simulink model "model"  (R2014a)
(part 4 of 6)

  bus259 : powerlib/Measurements/Load Flow Bus  LConnTagsString=a  ID=bus259  Vbase=440000  Vref=1  Vangle=0  VLF=1  angleLF=0
      settings: AttributesFormatString=|
      | %<ID>
      | %<Vbase>V
      | %<VLF>pu
      | %<angleLF>deg.
      | %<Name>
  bus26 : powerlib/Measurements/Load Flow Bus  LConnTagsString=a  ID=bus26  Vbase=138000  Vref=1  Vangle=0  VLF=1  angleLF=0
      settings: AttributesFormatString=|
      | %<ID>
      | %<Vbase>V
      | %<VLF>pu
      | %<angleLF>deg.
      | %<Name>
  bus260 : powerlib/Measurements/Load Flow Bus  LConnTagsString=a  ID=bus260  Vbase=440000  Vref=1  Vangle=0  VLF=1  angleLF=0
      settings: AttributesFormatString=|
      | %<ID>
      | %<Vbase>V
      | %<VLF>pu
      | %<angleLF>deg.
      | %<Name>
  bus261 : powerlib/Measurements/Load Flow Bus  LConnTagsString=a  ID=bus261  Vbase=440000  Vref=1  Vangle=0  VLF=1  angleLF=0
      settings: AttributesFormatString=|
      | %<ID>
      | %<Vbase>V
      | %<VLF>pu
      | %<angleLF>deg.
      | %<Name>
  bus262 : powerlib/Measurements/Load Flow Bus  LConnTagsString=a  ID=bus262  Vbase=500000  Vref=1  Vangle=0  VLF=1  angleLF=0
      settings: AttributesFormatString=|
      | %<ID>
      | %<Vbase>V
      | %<VLF>pu
      | %<angleLF>deg.
      | %<Name>
  bus263 : powerlib/Measurements/Load Flow Bus  LConnTagsString=a  ID=bus263  Vbase=500000  Vref=1  Vangle=0  VLF=1  angleLF=0
      settings: AttributesFormatString=|
      | %<ID>
      | %<Vbase>V
      | %<VLF>pu
      | %<angleLF>deg.
      | %<Name>
  bus264 : powerlib/Measurements/Load Flow Bus  LConnTagsString=a  ID=bus264  Vbase=500000  Vref=1  Vangle=0  VLF=1  angleLF=0
      settings: AttributesFormatString=|
      | %<ID>
      | %<Vbase>V
      | %<VLF>pu
      | %<angleLF>deg.
      | %<Name>
  bus265 : powerlib/Measurements/Load Flow Bus  LConnTagsString=a  ID=bus265  Vbase=500000  Vref=1  Vangle=0  VLF=1  angleLF=0
      settings: AttributesFormatString=|
      | %<ID>
      | %<Vbase>V
      | %<VLF>pu
      | %<angleLF>deg.
      | %<Name>
  bus266 : powerlib/Measurements/Load Flow Bus  LConnTagsString=a  ID=bus266  Vbase=500000  Vref=1  Vangle=0  VLF=1  angleLF=0
      settings: AttributesFormatString=|
      | %<ID>
      | %<Vbase>V
      | %<VLF>pu
      | %<angleLF>deg.
      | %<Name>
  bus267 : powerlib/Measurements/Load Flow Bus  LConnTagsString=a  ID=bus267  Vbase=500000  Vref=1  Vangle=0  VLF=1  angleLF=0
      settings: AttributesFormatString=|
      | %<ID>
      | %<Vbase>V
      | %<VLF>pu
      | %<angleLF>deg.
      | %<Name>
  bus268 : powerlib/Measurements/Load Flow Bus  LConnTagsString=a  ID=bus268  Vbase=500000  Vref=1  Vangle=0  VLF=1  angleLF=0
      settings: AttributesFormatString=|
      | %<ID>
      | %<Vbase>V
      | %<VLF>pu
      | %<angleLF>deg.
      | %<Name>
  bus269 : powerlib/Measurements/Load Flow Bus  LConnTagsString=a  ID=bus269  Vbase=500000  Vref=1  Vangle=0  VLF=1  angleLF=0
      settings: AttributesFormatString=|
      | %<ID>
      | %<Vbase>V
      | %<VLF>pu
      | %<angleLF>deg.
      | %<Name>
  bus27 : powerlib/Measurements/Load Flow Bus  LConnTagsString=a  ID=bus27  Vbase=138000  Vref=1  Vangle=0  VLF=1  angleLF=0
      settings: AttributesFormatString=|
      | %<ID>
      | %<Vbase>V
      | %<VLF>pu
      | %<angleLF>deg.
      | %<Name>
  bus270 : powerlib/Measurements/Load Flow Bus  LConnTagsString=a  ID=bus270  Vbase=500000  Vref=1  Vangle=0  VLF=1  angleLF=0
      settings: AttributesFormatString=|
      | %<ID>
      | %<Vbase>V
      | %<VLF>pu
      | %<angleLF>deg.
      | %<Name>
  bus271 : powerlib/Measurements/Load Flow Bus  LConnTagsString=a  ID=bus271  Vbase=500000  Vref=1  Vangle=0  VLF=1  angleLF=0
      settings: AttributesFormatString=|
      | %<ID>
      | %<Vbase>V
      | %<VLF>pu
      | %<angleLF>deg.
      | %<Name>
  bus272 : powerlib/Measurements/Load Flow Bus  LConnTagsString=a  ID=bus272  Vbase=500000  Vref=1  Vangle=0  VLF=1  angleLF=0
      settings: AttributesFormatString=|
      | %<ID>
      | %<Vbase>V
      | %<VLF>pu
      | %<angleLF>deg.
      | %<Name>
  bus273 : powerlib/Measurements/Load Flow Bus  LConnTagsString=a  ID=bus273  Vbase=500000  Vref=1  Vangle=0  VLF=1  angleLF=0
      settings: AttributesFormatString=|
      | %<ID>
      | %<Vbase>V
      | %<VLF>pu
      | %<angleLF>deg.
      | %<Name>
  bus274 : powerlib/Measurements/Load Flow Bus  LConnTagsString=a  ID=bus274  Vbase=500000  Vref=1  Vangle=0  VLF=1  angleLF=0
      settings: AttributesFormatString=|
      | %<ID>
      | %<Vbase>V
      | %<VLF>pu
      | %<angleLF>deg.
      | %<Name>
  bus275 : powerlib/Measurements/Load Flow Bus  LConnTagsString=a  ID=bus275  Vbase=500000  Vref=1  Vangle=0  VLF=1  angleLF=0
      settings: AttributesFormatString=|
      | %<ID>
      | %<Vbase>V
      | %<VLF>pu
      | %<angleLF>deg.
      | %<Name>
  bus276 : powerlib/Measurements/Load Flow Bus  LConnTagsString=a  ID=bus276  Vbase=500000  Vref=1  Vangle=0  VLF=1  angleLF=0
      settings: AttributesFormatString=|
      | %<ID>
      | %<Vbase>V
      | %<VLF>pu
      | %<angleLF>deg.
      | %<Name>
  bus277 : powerlib/Measurements/Load Flow Bus  LConnTagsString=a  ID=bus277  Vbase=500000  Vref=1  Vangle=0  VLF=1  angleLF=0
      settings: AttributesFormatString=|
      | %<ID>
      | %<Vbase>V
      | %<VLF>pu
      | %<angleLF>deg.
      | %<Name>
  bus278 : powerlib/Measurements/Load Flow Bus  LConnTagsString=a  ID=bus278  Vbase=500000  Vref=1  Vangle=0  VLF=1  angleLF=0
      settings: AttributesFormatString=|
      | %<ID>
      | %<Vbase>V
      | %<VLF>pu
      | %<angleLF>deg.
      | %<Name>
  bus279 : powerlib/Measurements/Load Flow Bus  LConnTagsString=a  ID=bus279  Vbase=500000  Vref=1  Vangle=0  VLF=1  angleLF=0
      settings: AttributesFormatString=|
      | %<ID>
      | %<Vbase>V
      | %<VLF>pu
      | %<angleLF>deg.
      | %<Name>
  bus28 : powerlib/Measurements/Load Flow Bus  LConnTagsString=a  ID=bus28  Vbase=138000  Vref=1  Vangle=0  VLF=1  angleLF=0
      settings: AttributesFormatString=|
      | %<ID>
      | %<Vbase>V
      | %<VLF>pu
      | %<angleLF>deg.
      | %<Name>
  bus280 : powerlib/Measurements/Load Flow Bus  LConnTagsString=a  ID=bus280  Vbase=500000  Vref=1  Vangle=0  VLF=1  angleLF=0
      settings: AttributesFormatString=|
      | %<ID>
      | %<Vbase>V
      | %<VLF>pu
      | %<angleLF>deg.
      | %<Name>
  bus281 : powerlib/Measurements/Load Flow Bus  LConnTagsString=a  ID=bus281  Vbase=500000  Vref=1  Vangle=0  VLF=1  angleLF=0
      settings: AttributesFormatString=|
      | %<ID>
      | %<Vbase>V
      | %<VLF>pu
      | %<angleLF>deg.
      | %<Name>
  bus282 : powerlib/Measurements/Load Flow Bus  LConnTagsString=a  ID=bus282  Vbase=500000  Vref=1  Vangle=0  VLF=1  angleLF=0
      settings: AttributesFormatString=|
      | %<ID>
      | %<Vbase>V
      | %<VLF>pu
      | %<angleLF>deg.
      | %<Name>
  bus283 : powerlib/Measurements/Load Flow Bus  LConnTagsString=a  ID=bus283  Vbase=500000  Vref=1  Vangle=0  VLF=1  angleLF=0
      settings: AttributesFormatString=|
      | %<ID>
      | %<Vbase>V
      | %<VLF>pu
      | %<angleLF>deg.
      | %<Name>
  bus284 : powerlib/Measurements/Load Flow Bus  LConnTagsString=a  ID=bus284  Vbase=500000  Vref=1  Vangle=0  VLF=1  angleLF=0
      settings: AttributesFormatString=|
      | %<ID>
      | %<Vbase>V
      | %<VLF>pu
      | %<angleLF>deg.
      | %<Name>
  bus285 : powerlib/Measurements/Load Flow Bus  LConnTagsString=a  ID=bus285  Vbase=500000  Vref=1  Vangle=0  VLF=1  angleLF=0
      settings: AttributesFormatString=|
      | %<ID>
      | %<Vbase>V
      | %<VLF>pu
      | %<angleLF>deg.
      | %<Name>
  bus286 : powerlib/Measurements/Load Flow Bus  LConnTagsString=a  ID=bus286  Vbase=500000  Vref=1  Vangle=0  VLF=1  angleLF=0
      settings: AttributesFormatString=|
      | %<ID>
      | %<Vbase>V
      | %<VLF>pu
      | %<angleLF>deg.
      | %<Name>
  bus287 : powerlib/Measurements/Load Flow Bus  LConnTagsString=a  ID=bus287  Vbase=500000  Vref=1  Vangle=0  VLF=1  angleLF=0
      settings: AttributesFormatString=|
      | %<ID>
      | %<Vbase>V
      | %<VLF>pu
      | %<angleLF>deg.
      | %<Name>
  bus288 : powerlib/Measurements/Load Flow Bus  LConnTagsString=a  ID=bus288  Vbase=500000  Vref=1  Vangle=0  VLF=1  angleLF=0
      settings: AttributesFormatString=|
      | %<ID>
      | %<Vbase>V
      | %<VLF>pu
      | %<angleLF>deg.
      | %<Name>
  bus289 : powerlib/Measurements/Load Flow Bus  LConnTagsString=a  ID=bus289  Vbase=500000  Vref=1  Vangle=0  VLF=1  angleLF=0
      settings: AttributesFormatString=|
      | %<ID>
      | %<Vbase>V
      | %<VLF>pu
      | %<angleLF>deg.
      | %<Name>
  bus29 : powerlib/Measurements/Load Flow Bus  LConnTagsString=a  ID=bus29  Vbase=138000  Vref=1  Vangle=0  VLF=1  angleLF=0
      settings: AttributesFormatString=|
      | %<ID>
      | %<Vbase>V
      | %<VLF>pu
      | %<angleLF>deg.
      | %<Name>
  bus290 : powerlib/Measurements/Load Flow Bus  LConnTagsString=a  ID=bus290  Vbase=500000  Vref=1  Vangle=0  VLF=1  angleLF=0
      settings: AttributesFormatString=|
      | %<ID>
      | %<Vbase>V
      | %<VLF>pu
      | %<angleLF>deg.
      | %<Name>
  bus291 : powerlib/Measurements/Load Flow Bus  LConnTagsString=a  ID=bus291  Vbase=500000  Vref=1  Vangle=0  VLF=1  angleLF=0
      settings: AttributesFormatString=|
      | %<ID>
      | %<Vbase>V
      | %<VLF>pu
      | %<angleLF>deg.
      | %<Name>
  bus292 : powerlib/Measurements/Load Flow Bus  LConnTagsString=a  ID=bus292  Vbase=500000  Vref=1  Vangle=0  VLF=1  angleLF=0
      settings: AttributesFormatString=|
      | %<ID>
      | %<Vbase>V
      | %<VLF>pu
      | %<angleLF>deg.
      | %<Name>
  bus293 : powerlib/Measurements/Load Flow Bus  LConnTagsString=a  ID=bus293  Vbase=500000  Vref=1  Vangle=0  VLF=1  angleLF=0
      settings: AttributesFormatString=|
      | %<ID>
      | %<Vbase>V
      | %<VLF>pu
      | %<angleLF>deg.
      | %<Name>
  bus294 : powerlib/Measurements/Load Flow Bus  LConnTagsString=a  ID=bus294  Vbase=500000  Vref=1  Vangle=0  VLF=1  angleLF=0
      settings: AttributesFormatString=|
      | %<ID>
      | %<Vbase>V
      | %<VLF>pu
      | %<angleLF>deg.
      | %<Name>
  bus295 : powerlib/Measurements/Load Flow Bus  LConnTagsString=a  ID=bus295  Vbase=500000  Vref=1  Vangle=0  VLF=1  angleLF=0
      settings: AttributesFormatString=|
      | %<ID>
      | %<Vbase>V
      | %<VLF>pu
      | %<angleLF>deg.
      | %<Name>
  bus296 : powerlib/Measurements/Load Flow Bus  LConnTagsString=a  ID=bus296  Vbase=500000  Vref=1  Vangle=0  VLF=1  angleLF=0
      settings: AttributesFormatString=|
      | %<ID>
      | %<Vbase>V
      | %<VLF>pu
      | %<angleLF>deg.
      | %<Name>
  bus297 : powerlib/Measurements/Load Flow Bus  LConnTagsString=a  ID=bus297  Vbase=500000  Vref=1  Vangle=0  VLF=1  angleLF=0
      settings: AttributesFormatString=|
      | %<ID>
      | %<Vbase>V
      | %<VLF>pu
      | %<angleLF>deg.
      | %<Name>
  bus298 : powerlib/Measurements/Load Flow Bus  LConnTagsString=a  ID=bus298  Vbase=500000  Vref=1  Vangle=0  VLF=1  angleLF=0
      settings: AttributesFormatString=|
      | %<ID>
      | %<Vbase>V
      | %<VLF>pu
      | %<angleLF>deg.
      | %<Name>
  bus299 : powerlib/Measurements/Load Flow Bus  LConnTagsString=a  ID=bus299  Vbase=500000  Vref=1  Vangle=0  VLF=1  angleLF=0
      settings: AttributesFormatString=|
      | %<ID>
      | %<Vbase>V
      | %<VLF>pu
      | %<angleLF>deg.
      | %<Name>
  bus3 : powerlib/Measurements/Load Flow Bus  LConnTagsString=a  ID=bus3  Vbase=138000  Vref=1  Vangle=0  VLF=1  angleLF=0
      settings: AttributesFormatString=|
      | %<ID>
      | %<Vbase>V
      | %<VLF>pu
      | %<angleLF>deg.
      | %<Name>
  bus30 : powerlib/Measurements/Load Flow Bus  LConnTagsString=a  ID=bus30  Vbase=138000  Vref=1  Vangle=0  VLF=1  angleLF=0
      settings: AttributesFormatString=|
      | %<ID>
      | %<Vbase>V
      | %<VLF>pu
      | %<angleLF>deg.
      | %<Name>
  bus300 : powerlib/Measurements/Load Flow Bus  LConnTagsString=a  ID=bus300  Vbase=500000  Vref=1  Vangle=0  VLF=1  angleLF=0
      settings: AttributesFormatString=|
      | %<ID>
      | %<Vbase>V
      | %<VLF>pu
      | %<angleLF>deg.
      | %<Name>
  bus301 : powerlib/Measurements/Load Flow Bus  LConnTagsString=a  ID=bus301  Vbase=500000  Vref=1  Vangle=0  VLF=1  angleLF=0
      settings: AttributesFormatString=|
      | %<ID>
      | %<Vbase>V
      | %<VLF>pu
      | %<angleLF>deg.
      | %<Name>
  bus302 : powerlib/Measurements/Load Flow Bus  LConnTagsString=a  ID=bus302  Vbase=500000  Vref=1  Vangle=0  VLF=1  angleLF=0
      settings: AttributesFormatString=|
      | %<ID>
      | %<Vbase>V
      | %<VLF>pu
      | %<angleLF>deg.
      | %<Name>
  bus303 : powerlib/Measurements/Load Flow Bus  LConnTagsString=a  ID=bus303  Vbase=500000  Vref=1  Vangle=0  VLF=1  angleLF=0
      settings: AttributesFormatString=|
      | %<ID>
      | %<Vbase>V
      | %<VLF>pu
      | %<angleLF>deg.
      | %<Name>
  bus304 : powerlib/Measurements/Load Flow Bus  LConnTagsString=a  ID=bus304  Vbase=500000  Vref=1  Vangle=0  VLF=1  angleLF=0
      settings: AttributesFormatString=|
      | %<ID>
      | %<Vbase>V
      | %<VLF>pu
      | %<angleLF>deg.
      | %<Name>
  bus305 : powerlib/Measurements/Load Flow Bus  LConnTagsString=a  ID=bus305  Vbase=500000  Vref=1  Vangle=0  VLF=1  angleLF=0
      settings: AttributesFormatString=|
      | %<ID>
      | %<Vbase>V
      | %<VLF>pu
      | %<angleLF>deg.
      | %<Name>
  bus306 : powerlib/Measurements/Load Flow Bus  LConnTagsString=a  ID=bus306  Vbase=500000  Vref=1  Vangle=0  VLF=1  angleLF=0
      settings: AttributesFormatString=|
      | %<ID>
      | %<Vbase>V
      | %<VLF>pu
      | %<angleLF>deg.
      | %<Name>
  bus307 : powerlib/Measurements/Load Flow Bus  LConnTagsString=a  ID=bus307  Vbase=500000  Vref=1  Vangle=0  VLF=1  angleLF=0
      settings: AttributesFormatString=|
      | %<ID>
      | %<Vbase>V
      | %<VLF>pu
      | %<angleLF>deg.
      | %<Name>
  bus308 : powerlib/Measurements/Load Flow Bus  LConnTagsString=a  ID=bus308  Vbase=500000  Vref=1  Vangle=0  VLF=1  angleLF=0
      settings: AttributesFormatString=|
      | %<ID>
      | %<Vbase>V
      | %<VLF>pu
      | %<angleLF>deg.
      | %<Name>
  bus309 : powerlib/Measurements/Load Flow Bus  LConnTagsString=a  ID=bus309  Vbase=500000  Vref=1  Vangle=0  VLF=1  angleLF=0
      settings: AttributesFormatString=|
      | %<ID>
      | %<Vbase>V
      | %<VLF>pu
      | %<angleLF>deg.
      | %<Name>
  bus31 : powerlib/Measurements/Load Flow Bus  LConnTagsString=a  ID=bus31  Vbase=138000  Vref=1  Vangle=0  VLF=1  angleLF=0
      settings: AttributesFormatString=|
      | %<ID>
      | %<Vbase>V
      | %<VLF>pu
      | %<angleLF>deg.
      | %<Name>
  bus310 : powerlib/Measurements/Load Flow Bus  LConnTagsString=a  ID=bus310  Vbase=500000  Vref=1  Vangle=0  VLF=1  angleLF=0
      settings: AttributesFormatString=|
      | %<ID>
      | %<Vbase>V
      | %<VLF>pu
      | %<angleLF>deg.
      | %<Name>
  bus311 : powerlib/Measurements/Load Flow Bus  LConnTagsString=a  ID=bus311  Vbase=500000  Vref=1  Vangle=0  VLF=1  angleLF=0
      settings: AttributesFormatString=|
      | %<ID>
      | %<Vbase>V
      | %<VLF>pu
      | %<angleLF>deg.
      | %<Name>
  bus312 : powerlib/Measurements/Load Flow Bus  LConnTagsString=a  ID=bus312  Vbase=500000  Vref=1  Vangle=0  VLF=1  angleLF=0
      settings: AttributesFormatString=|
      | %<ID>
      | %<Vbase>V
      | %<VLF>pu
      | %<angleLF>deg.
      | %<Name>
  bus313 : powerlib/Measurements/Load Flow Bus  LConnTagsString=a  ID=bus313  Vbase=500000  Vref=1  Vangle=0  VLF=1  angleLF=0
      settings: AttributesFormatString=|
      | %<ID>
      | %<Vbase>V
      | %<VLF>pu
      | %<angleLF>deg.
      | %<Name>
  bus314 : powerlib/Measurements/Load Flow Bus  LConnTagsString=a  ID=bus314  Vbase=500000  Vref=1  Vangle=0  VLF=1  angleLF=0
      settings: AttributesFormatString=|
      | %<ID>
      | %<Vbase>V
      | %<VLF>pu
      | %<angleLF>deg.
      | %<Name>
  bus315 : powerlib/Measurements/Load Flow Bus  LConnTagsString=a  ID=bus315  Vbase=500000  Vref=1  Vangle=0  VLF=1  angleLF=0
      settings: AttributesFormatString=|
      | %<ID>
      | %<Vbase>V
      | %<VLF>pu
      | %<angleLF>deg.
      | %<Name>
  bus316 : powerlib/Measurements/Load Flow Bus  LConnTagsString=a  ID=bus316  Vbase=500000  Vref=1  Vangle=0  VLF=1  angleLF=0
      settings: AttributesFormatString=|
      | %<ID>
      | %<Vbase>V
      | %<VLF>pu
      | %<angleLF>deg.
      | %<Name>
  bus317 : powerlib/Measurements/Load Flow Bus  LConnTagsString=a  ID=bus317  Vbase=500000  Vref=1  Vangle=0  VLF=1  angleLF=0
      settings: AttributesFormatString=|
      | %<ID>
      | %<Vbase>V
      | %<VLF>pu
      | %<angleLF>deg.
      | %<Name>
  bus318 : powerlib/Measurements/Load Flow Bus  LConnTagsString=a  ID=bus318  Vbase=500000  Vref=1  Vangle=0  VLF=1  angleLF=0
      settings: AttributesFormatString=|
      | %<ID>
      | %<Vbase>V
      | %<VLF>pu
      | %<angleLF>deg.
      | %<Name>
  bus319 : powerlib/Measurements/Load Flow Bus  LConnTagsString=a  ID=bus319  Vbase=500000  Vref=1  Vangle=0  VLF=1  angleLF=0
      settings: AttributesFormatString=|
      | %<ID>
      | %<Vbase>V
      | %<VLF>pu
      | %<angleLF>deg.
      | %<Name>
  bus32 : powerlib/Measurements/Load Flow Bus  LConnTagsString=a  ID=bus32  Vbase=138000  Vref=1  Vangle=0  VLF=1  angleLF=0
      settings: AttributesFormatString=|
      | %<ID>
      | %<Vbase>V
      | %<VLF>pu
      | %<angleLF>deg.
      | %<Name>
  bus320 : powerlib/Measurements/Load Flow Bus  LConnTagsString=a  ID=bus320  Vbase=500000  Vref=1  Vangle=0  VLF=1  angleLF=0
      settings: AttributesFormatString=|
      | %<ID>
      | %<Vbase>V
      | %<VLF>pu
      | %<angleLF>deg.
      | %<Name>
  bus321 : powerlib/Measurements/Load Flow Bus  LConnTagsString=a  ID=bus321  Vbase=500000  Vref=1  Vangle=0  VLF=1  angleLF=0
      settings: AttributesFormatString=|
      | %<ID>
      | %<Vbase>V
      | %<VLF>pu
      | %<angleLF>deg.
      | %<Name>
  bus322 : powerlib/Measurements/Load Flow Bus  LConnTagsString=a  ID=bus322  Vbase=500000  Vref=1  Vangle=0  VLF=1  angleLF=0
      settings: AttributesFormatString=|
      | %<ID>
      | %<Vbase>V
      | %<VLF>pu
      | %<angleLF>deg.
      | %<Name>
  bus323 : powerlib/Measurements/Load Flow Bus  LConnTagsString=a  ID=bus323  Vbase=500000  Vref=1  Vangle=0  VLF=1  angleLF=0
      settings: AttributesFormatString=|
      | %<ID>
      | %<Vbase>V
      | %<VLF>pu
      | %<angleLF>deg.
      | %<Name>
  bus324 : powerlib/Measurements/Load Flow Bus  LConnTagsString=a  ID=bus324  Vbase=500000  Vref=1  Vangle=0  VLF=1  angleLF=0
      settings: AttributesFormatString=|
      | %<ID>
      | %<Vbase>V
      | %<VLF>pu
      | %<angleLF>deg.
      | %<Name>
  bus325 : powerlib/Measurements/Load Flow Bus  LConnTagsString=a  ID=bus325  Vbase=500000  Vref=1  Vangle=0  VLF=1  angleLF=0
      settings: AttributesFormatString=|
      | %<ID>
      | %<Vbase>V
      | %<VLF>pu
      | %<angleLF>deg.
      | %<Name>
  bus326 : powerlib/Measurements/Load Flow Bus  LConnTagsString=a  ID=bus326  Vbase=500000  Vref=1  Vangle=0  VLF=1  angleLF=0
      settings: AttributesFormatString=|
      | %<ID>
      | %<Vbase>V
      | %<VLF>pu
      | %<angleLF>deg.
      | %<Name>
  bus327 : powerlib/Measurements/Load Flow Bus  LConnTagsString=a  ID=bus327  Vbase=500000  Vref=1  Vangle=0  VLF=1  angleLF=0
      settings: AttributesFormatString=|
      | %<ID>
      | %<Vbase>V
      | %<VLF>pu
      | %<angleLF>deg.
      | %<Name>
  bus328 : powerlib/Measurements/Load Flow Bus  LConnTagsString=a  ID=bus328  Vbase=500000  Vref=1  Vangle=0  VLF=1  angleLF=0
      settings: AttributesFormatString=|
      | %<ID>
      | %<Vbase>V
      | %<VLF>pu
      | %<angleLF>deg.
      | %<Name>
  bus329 : powerlib/Measurements/Load Flow Bus  LConnTagsString=a  ID=bus329  Vbase=500000  Vref=1  Vangle=0  VLF=1  angleLF=0
      settings: AttributesFormatString=|
      | %<ID>
      | %<Vbase>V
      | %<VLF>pu
      | %<angleLF>deg.
      | %<Name>
  bus33 : powerlib/Measurements/Load Flow Bus  LConnTagsString=a  ID=bus33  Vbase=138000  Vref=1  Vangle=0  VLF=1  angleLF=0
      settings: AttributesFormatString=|
      | %<ID>
      | %<Vbase>V
      | %<VLF>pu
      | %<angleLF>deg.
      | %<Name>
  bus330 : powerlib/Measurements/Load Flow Bus  LConnTagsString=a  ID=bus330  Vbase=500000  Vref=1  Vangle=0  VLF=1  angleLF=0
      settings: AttributesFormatString=|
      | %<ID>
      | %<Vbase>V
      | %<VLF>pu
      | %<angleLF>deg.
      | %<Name>
  bus331 : powerlib/Measurements/Load Flow Bus  LConnTagsString=a  ID=bus331  Vbase=500000  Vref=1  Vangle=0  VLF=1  angleLF=0
      settings: AttributesFormatString=|
      | %<ID>
      | %<Vbase>V
      | %<VLF>pu
      | %<angleLF>deg.
      | %<Name>
  bus332 : powerlib/Measurements/Load Flow Bus  LConnTagsString=a  ID=bus332  Vbase=500000  Vref=1  Vangle=0  VLF=1  angleLF=0
      settings: AttributesFormatString=|
      | %<ID>
      | %<Vbase>V
      | %<VLF>pu
      | %<angleLF>deg.
      | %<Name>
  bus333 : powerlib/Measurements/Load Flow Bus  LConnTagsString=a  ID=bus333  Vbase=500000  Vref=1  Vangle=0  VLF=1  angleLF=0
      settings: AttributesFormatString=|
      | %<ID>
      | %<Vbase>V
      | %<VLF>pu
      | %<angleLF>deg.
      | %<Name>
  bus334 : powerlib/Measurements/Load Flow Bus  LConnTagsString=a  ID=bus334  Vbase=500000  Vref=1  Vangle=0  VLF=1  angleLF=0
      settings: AttributesFormatString=|
      | %<ID>
      | %<Vbase>V
      | %<VLF>pu
      | %<angleLF>deg.
      | %<Name>
  bus335 : powerlib/Measurements/Load Flow Bus  LConnTagsString=a  ID=bus335  Vbase=500000  Vref=1  Vangle=0  VLF=1  angleLF=0
      settings: AttributesFormatString=|
      | %<ID>
      | %<Vbase>V
      | %<VLF>pu
      | %<angleLF>deg.
      | %<Name>
  bus336 : powerlib/Measurements/Load Flow Bus  LConnTagsString=a  ID=bus336  Vbase=500000  Vref=1  Vangle=0  VLF=1  angleLF=0
      settings: AttributesFormatString=|
      | %<ID>
      | %<Vbase>V
      | %<VLF>pu
      | %<angleLF>deg.
      | %<Name>
  bus337 : powerlib/Measurements/Load Flow Bus  LConnTagsString=a  ID=bus337  Vbase=500000  Vref=1  Vangle=0  VLF=1  angleLF=0
      settings: AttributesFormatString=|
      | %<ID>
      | %<Vbase>V
      | %<VLF>pu
      | %<angleLF>deg.
      | %<Name>
  bus338 : powerlib/Measurements/Load Flow Bus  LConnTagsString=a  ID=bus338  Vbase=500000  Vref=1  Vangle=0  VLF=1  angleLF=0
      settings: AttributesFormatString=|
      | %<ID>
      | %<Vbase>V
      | %<VLF>pu
      | %<angleLF>deg.
      | %<Name>
  bus339 : powerlib/Measurements/Load Flow Bus  LConnTagsString=a  ID=bus339  Vbase=500000  Vref=1  Vangle=0  VLF=1  angleLF=0
      settings: AttributesFormatString=|
      | %<ID>
      | %<Vbase>V
      | %<VLF>pu
      | %<angleLF>deg.
      | %<Name>
  bus34 : powerlib/Measurements/Load Flow Bus  LConnTagsString=a  ID=bus34  Vbase=138000  Vref=1  Vangle=0  VLF=1  angleLF=0
      settings: AttributesFormatString=|
      | %<ID>
      | %<Vbase>V
      | %<VLF>pu
      | %<angleLF>deg.
      | %<Name>
  bus340 : powerlib/Measurements/Load Flow Bus  LConnTagsString=a  ID=bus340  Vbase=500000  Vref=1  Vangle=0  VLF=1  angleLF=0
      settings: AttributesFormatString=|
      | %<ID>
      | %<Vbase>V
      | %<VLF>pu
      | %<angleLF>deg.
      | %<Name>
  bus341 : powerlib/Measurements/Load Flow Bus  LConnTagsString=a  ID=bus341  Vbase=500000  Vref=1  Vangle=0  VLF=1  angleLF=0
      settings: AttributesFormatString=|
      | %<ID>
      | %<Vbase>V
      | %<VLF>pu
      | %<angleLF>deg.
      | %<Name>
  bus342 : powerlib/Measurements/Load Flow Bus  LConnTagsString=a  ID=bus342  Vbase=500000  Vref=1  Vangle=0  VLF=1  angleLF=0
      settings: AttributesFormatString=|
      | %<ID>
      | %<Vbase>V
      | %<VLF>pu
      | %<angleLF>deg.
      | %<Name>
  bus343 : powerlib/Measurements/Load Flow Bus  LConnTagsString=a  ID=bus343  Vbase=500000  Vref=1  Vangle=0  VLF=1  angleLF=0
      settings: AttributesFormatString=|
      | %<ID>
      | %<Vbase>V
      | %<VLF>pu
      | %<angleLF>deg.
      | %<Name>
  bus344 : powerlib/Measurements/Load Flow Bus  LConnTagsString=a  ID=bus344  Vbase=500000  Vref=1  Vangle=0  VLF=1  angleLF=0
      settings: AttributesFormatString=|
      | %<ID>
      | %<Vbase>V
      | %<VLF>pu
      | %<angleLF>deg.
      | %<Name>
  bus345 : powerlib/Measurements/Load Flow Bus  LConnTagsString=a  ID=bus345  Vbase=500000  Vref=1  Vangle=0  VLF=1  angleLF=0
      settings: AttributesFormatString=|
      | %<ID>
      | %<Vbase>V
      | %<VLF>pu
      | %<angleLF>deg.
      | %<Name>
  bus346 : powerlib/Measurements/Load Flow Bus  LConnTagsString=a  ID=bus346  Vbase=500000  Vref=1  Vangle=0  VLF=1  angleLF=0
      settings: AttributesFormatString=|
      | %<ID>
      | %<Vbase>V
      | %<VLF>pu
      | %<angleLF>deg.
      | %<Name>
  bus347 : powerlib/Measurements/Load Flow Bus  LConnTagsString=a  ID=bus347  Vbase=500000  Vref=1  Vangle=0  VLF=1  angleLF=0
      settings: AttributesFormatString=|
      | %<ID>
      | %<Vbase>V
      | %<VLF>pu
      | %<angleLF>deg.
      | %<Name>
  bus348 : powerlib/Measurements/Load Flow Bus  LConnTagsString=a  ID=bus348  Vbase=500000  Vref=1  Vangle=0  VLF=1  angleLF=0
      settings: AttributesFormatString=|
      | %<ID>
      | %<Vbase>V
      | %<VLF>pu
      | %<angleLF>deg.
      | %<Name>
  bus349 : powerlib/Measurements/Load Flow Bus  LConnTagsString=a  ID=bus349  Vbase=750000  Vref=1  Vangle=0  VLF=1  angleLF=0
      settings: AttributesFormatString=|
      | %<ID>
      | %<Vbase>V
      | %<VLF>pu
      | %<angleLF>deg.
      | %<Name>
  bus35 : powerlib/Measurements/Load Flow Bus  LConnTagsString=a  ID=bus35  Vbase=138000  Vref=1  Vangle=0  VLF=1  angleLF=0
      settings: AttributesFormatString=|
      | %<ID>
      | %<Vbase>V
      | %<VLF>pu
      | %<angleLF>deg.
      | %<Name>
  bus350 : powerlib/Measurements/Load Flow Bus  LConnTagsString=a  ID=bus350  Vbase=750000  Vref=1  Vangle=0  VLF=1  angleLF=0
      settings: AttributesFormatString=|
      | %<ID>
      | %<Vbase>V
      | %<VLF>pu
      | %<angleLF>deg.
      | %<Name>
  bus351 : powerlib/Measurements/Load Flow Bus  LConnTagsString=a  ID=bus351  Vbase=750000  Vref=1  Vangle=0  VLF=1  angleLF=0
      settings: AttributesFormatString=|
      | %<ID>
      | %<Vbase>V
      | %<VLF>pu
      | %<angleLF>deg.
      | %<Name>
  bus352 : powerlib/Measurements/Load Flow Bus  LConnTagsString=a  ID=bus352  Vbase=750000  Vref=1  Vangle=0  VLF=1  angleLF=0
      settings: AttributesFormatString=|
      | %<ID>
      | %<Vbase>V
      | %<VLF>pu
      | %<angleLF>deg.
      | %<Name>
  bus353 : powerlib/Measurements/Load Flow Bus  LConnTagsString=a  ID=bus353  Vbase=138000  Vref=1  Vangle=0  VLF=1  angleLF=0
      settings: AttributesFormatString=|
      | %<ID>
      | %<Vbase>V
      | %<VLF>pu
      | %<angleLF>deg.
      | %<Name>
  bus354 : powerlib/Measurements/Load Flow Bus  LConnTagsString=a  ID=bus354  Vbase=138000  Vref=1  Vangle=0  VLF=1  angleLF=0
      settings: AttributesFormatString=|
      | %<ID>
      | %<Vbase>V
      | %<VLF>pu
      | %<angleLF>deg.
      | %<Name>
  bus355 : powerlib/Measurements/Load Flow Bus  LConnTagsString=a  ID=bus355  Vbase=138000  Vref=1  Vangle=0  VLF=1  angleLF=0
      settings: AttributesFormatString=|
      | %<ID>
      | %<Vbase>V
      | %<VLF>pu
      | %<angleLF>deg.
      | %<Name>
  bus356 : powerlib/Measurements/Load Flow Bus  LConnTagsString=a  ID=bus356  Vbase=138000  Vref=1  Vangle=0  VLF=1  angleLF=0
      settings: AttributesFormatString=|
      | %<ID>
      | %<Vbase>V
      | %<VLF>pu
      | %<angleLF>deg.
      | %<Name>
  bus357 : powerlib/Measurements/Load Flow Bus  LConnTagsString=a  ID=bus357  Vbase=138000  Vref=1  Vangle=0  VLF=1  angleLF=0
      settings: AttributesFormatString=|
      | %<ID>
      | %<Vbase>V
      | %<VLF>pu
      | %<angleLF>deg.
      | %<Name>
  bus358 : powerlib/Measurements/Load Flow Bus  LConnTagsString=a  ID=bus358  Vbase=138000  Vref=1  Vangle=0  VLF=1  angleLF=0
      settings: AttributesFormatString=|
      | %<ID>
      | %<Vbase>V
      | %<VLF>pu
      | %<angleLF>deg.
      | %<Name>
  bus359 : powerlib/Measurements/Load Flow Bus  LConnTagsString=a  ID=bus359  Vbase=138000  Vref=1  Vangle=0  VLF=1  angleLF=0
      settings: AttributesFormatString=|
      | %<ID>
      | %<Vbase>V
      | %<VLF>pu
      | %<angleLF>deg.
      | %<Name>
  bus36 : powerlib/Measurements/Load Flow Bus  LConnTagsString=a  ID=bus36  Vbase=138000  Vref=1  Vangle=0  VLF=1  angleLF=0
      settings: AttributesFormatString=|
      | %<ID>
      | %<Vbase>V
      | %<VLF>pu
      | %<angleLF>deg.
      | %<Name>
  bus360 : powerlib/Measurements/Load Flow Bus  LConnTagsString=a  ID=bus360  Vbase=138000  Vref=1  Vangle=0  VLF=1  angleLF=0
      settings: AttributesFormatString=|
      | %<ID>
      | %<Vbase>V
      | %<VLF>pu
      | %<angleLF>deg.
      | %<Name>
  bus361 : powerlib/Measurements/Load Flow Bus  LConnTagsString=a  ID=bus361  Vbase=138000  Vref=1  Vangle=0  VLF=1  angleLF=0
      settings: AttributesFormatString=|
      | %<ID>
      | %<Vbase>V
      | %<VLF>pu
      | %<angleLF>deg.
      | %<Name>
  bus362 : powerlib/Measurements/Load Flow Bus  LConnTagsString=a  ID=bus362  Vbase=138000  Vref=1  Vangle=0  VLF=1  angleLF=0
      settings: AttributesFormatString=|
      | %<ID>
      | %<Vbase>V
      | %<VLF>pu
      | %<angleLF>deg.
      | %<Name>
  bus363 : powerlib/Measurements/Load Flow Bus  LConnTagsString=a  ID=bus363  Vbase=138000  Vref=1  Vangle=0  VLF=1  angleLF=0
      settings: AttributesFormatString=|
      | %<ID>
      | %<Vbase>V
      | %<VLF>pu
      | %<angleLF>deg.
      | %<Name>
  bus364 : powerlib/Measurements/Load Flow Bus  LConnTagsString=a  ID=bus364  Vbase=138000  Vref=1  Vangle=0  VLF=1  angleLF=0
      settings: AttributesFormatString=|
      | %<ID>
      | %<Vbase>V
      | %<VLF>pu
      | %<angleLF>deg.
      | %<Name>
  bus365 : powerlib/Measurements/Load Flow Bus  LConnTagsString=a  ID=bus365  Vbase=138000  Vref=1  Vangle=0  VLF=1  angleLF=0
      settings: AttributesFormatString=|
      | %<ID>
      | %<Vbase>V
      | %<VLF>pu
      | %<angleLF>deg.
      | %<Name>
  bus366 : powerlib/Measurements/Load Flow Bus  LConnTagsString=a  ID=bus366  Vbase=138000  Vref=1  Vangle=0  VLF=1  angleLF=0
      settings: AttributesFormatString=|
      | %<ID>
      | %<Vbase>V
      | %<VLF>pu
      | %<angleLF>deg.
      | %<Name>
  bus367 : powerlib/Measurements/Load Flow Bus  LConnTagsString=a  ID=bus367  Vbase=138000  Vref=1  Vangle=0  VLF=1  angleLF=0
      settings: AttributesFormatString=|
      | %<ID>
      | %<Vbase>V
      | %<VLF>pu
      | %<angleLF>deg.
      | %<Name>
  bus368 : powerlib/Measurements/Load Flow Bus  LConnTagsString=a  ID=bus368  Vbase=138000  Vref=1  Vangle=0  VLF=1  angleLF=0
      settings: AttributesFormatString=|
      | %<ID>
      | %<Vbase>V
      | %<VLF>pu
      | %<angleLF>deg.
      | %<Name>
  bus369 : powerlib/Measurements/Load Flow Bus  LConnTagsString=a  ID=bus369  Vbase=138000  Vref=1  Vangle=0  VLF=1  angleLF=0
      settings: AttributesFormatString=|
      | %<ID>
      | %<Vbase>V
      | %<VLF>pu
      | %<angleLF>deg.
      | %<Name>
  bus37 : powerlib/Measurements/Load Flow Bus  LConnTagsString=a  ID=bus37  Vbase=138000  Vref=1  Vangle=0  VLF=1  angleLF=0
      settings: AttributesFormatString=|
      | %<ID>
      | %<Vbase>V
      | %<VLF>pu
      | %<angleLF>deg.
      | %<Name>
  bus370 : powerlib/Measurements/Load Flow Bus  LConnTagsString=a  ID=bus370  Vbase=138000  Vref=1  Vangle=0  VLF=1  angleLF=0
      settings: AttributesFormatString=|
      | %<ID>
      | %<Vbase>V
      | %<VLF>pu
      | %<angleLF>deg.
      | %<Name>
  bus371 : powerlib/Measurements/Load Flow Bus  LConnTagsString=a  ID=bus371  Vbase=138000  Vref=1  Vangle=0  VLF=1  angleLF=0
      settings: AttributesFormatString=|
      | %<ID>
      | %<Vbase>V
      | %<VLF>pu
      | %<angleLF>deg.
      | %<Name>
  bus372 : powerlib/Measurements/Load Flow Bus  LConnTagsString=a  ID=bus372  Vbase=138000  Vref=1  Vangle=0  VLF=1  angleLF=0
      settings: AttributesFormatString=|
      | %<ID>
      | %<Vbase>V
      | %<VLF>pu
      | %<angleLF>deg.
      | %<Name>
  bus373 : powerlib/Measurements/Load Flow Bus  LConnTagsString=a  ID=bus373  Vbase=138000  Vref=1  Vangle=0  VLF=1  angleLF=0
      settings: AttributesFormatString=|
      | %<ID>
      | %<Vbase>V
      | %<VLF>pu
      | %<angleLF>deg.
      | %<Name>
  bus374 : powerlib/Measurements/Load Flow Bus  LConnTagsString=a  ID=bus374  Vbase=138000  Vref=1  Vangle=0  VLF=1  angleLF=0
      settings: AttributesFormatString=|
      | %<ID>
      | %<Vbase>V
      | %<VLF>pu
      | %<angleLF>deg.
      | %<Name>
  bus375 : powerlib/Measurements/Load Flow Bus  LConnTagsString=a  ID=bus375  Vbase=138000  Vref=1  Vangle=0  VLF=1  angleLF=0
      settings: AttributesFormatString=|
      | %<ID>
      | %<Vbase>V
      | %<VLF>pu
      | %<angleLF>deg.
      | %<Name>
  bus376 : powerlib/Measurements/Load Flow Bus  LConnTagsString=a  ID=bus376  Vbase=138000  Vref=1  Vangle=0  VLF=1  angleLF=0
      settings: AttributesFormatString=|
      | %<ID>
      | %<Vbase>V
      | %<VLF>pu
      | %<angleLF>deg.
      | %<Name>
  bus377 : powerlib/Measurements/Load Flow Bus  LConnTagsString=a  ID=bus377  Vbase=138000  Vref=1  Vangle=0  VLF=1  angleLF=0
      settings: AttributesFormatString=|
      | %<ID>
      | %<Vbase>V
      | %<VLF>pu
      | %<angleLF>deg.
      | %<Name>
  bus378 : powerlib/Measurements/Load Flow Bus  LConnTagsString=a  ID=bus378  Vbase=138000  Vref=1  Vangle=0  VLF=1  angleLF=0
      settings: AttributesFormatString=|
      | %<ID>
      | %<Vbase>V
      | %<VLF>pu
      | %<angleLF>deg.
      | %<Name>
  bus379 : powerlib/Measurements/Load Flow Bus  LConnTagsString=a  ID=bus379  Vbase=138000  Vref=1  Vangle=0  VLF=1  angleLF=0
      settings: AttributesFormatString=|
      | %<ID>
      | %<Vbase>V
      | %<VLF>pu
      | %<angleLF>deg.
      | %<Name>
  bus38 : powerlib/Measurements/Load Flow Bus  LConnTagsString=a  ID=bus38  Vbase=138000  Vref=1  Vangle=0  VLF=1  angleLF=0
      settings: AttributesFormatString=|
      | %<ID>
      | %<Vbase>V
      | %<VLF>pu
      | %<angleLF>deg.
      | %<Name>
  bus380 : powerlib/Measurements/Load Flow Bus  LConnTagsString=a  ID=bus380  Vbase=138000  Vref=1  Vangle=0  VLF=1  angleLF=0
      settings: AttributesFormatString=|
      | %<ID>
      | %<Vbase>V
      | %<VLF>pu
      | %<angleLF>deg.
      | %<Name>
  bus381 : powerlib/Measurements/Load Flow Bus  LConnTagsString=a  ID=bus381  Vbase=138000  Vref=1  Vangle=0  VLF=1  angleLF=0
      settings: AttributesFormatString=|
      | %<ID>
      | %<Vbase>V
      | %<VLF>pu
      | %<angleLF>deg.
      | %<Name>
  bus382 : powerlib/Measurements/Load Flow Bus  LConnTagsString=a  ID=bus382  Vbase=138000  Vref=1  Vangle=0  VLF=1  angleLF=0
      settings: AttributesFormatString=|
      | %<ID>
      | %<Vbase>V
      | %<VLF>pu
      | %<angleLF>deg.
      | %<Name>
  bus383 : powerlib/Measurements/Load Flow Bus  LConnTagsString=a  ID=bus383  Vbase=138000  Vref=1  Vangle=0  VLF=1  angleLF=0
      settings: AttributesFormatString=|
      | %<ID>
      | %<Vbase>V
      | %<VLF>pu
      | %<angleLF>deg.
      | %<Name>
  bus384 : powerlib/Measurements/Load Flow Bus  LConnTagsString=a  ID=bus384  Vbase=138000  Vref=1  Vangle=0  VLF=1  angleLF=0
      settings: AttributesFormatString=|
      | %<ID>
      | %<Vbase>V
      | %<VLF>pu
      | %<angleLF>deg.
      | %<Name>
  bus385 : powerlib/Measurements/Load Flow Bus  LConnTagsString=a  ID=bus385  Vbase=138000  Vref=1  Vangle=0  VLF=1  angleLF=0
      settings: AttributesFormatString=|
      | %<ID>
      | %<Vbase>V
      | %<VLF>pu
      | %<angleLF>deg.
      | %<Name>
  bus386 : powerlib/Measurements/Load Flow Bus  LConnTagsString=a  ID=bus386  Vbase=138000  Vref=1  Vangle=0  VLF=1  angleLF=0
      settings: AttributesFormatString=|
      | %<ID>
      | %<Vbase>V
      | %<VLF>pu
      | %<angleLF>deg.
      | %<Name>
  bus387 : powerlib/Measurements/Load Flow Bus  LConnTagsString=a  ID=bus387  Vbase=138000  Vref=1  Vangle=0  VLF=1  angleLF=0
      settings: AttributesFormatString=|
      | %<ID>
      | %<Vbase>V
      | %<VLF>pu
      | %<angleLF>deg.
      | %<Name>
  bus388 : powerlib/Measurements/Load Flow Bus  LConnTagsString=a  ID=bus388  Vbase=138000  Vref=1  Vangle=0  VLF=1  angleLF=0
      settings: AttributesFormatString=|
      | %<ID>
      | %<Vbase>V
      | %<VLF>pu
      | %<angleLF>deg.
      | %<Name>
  bus389 : powerlib/Measurements/Load Flow Bus  LConnTagsString=a  ID=bus389  Vbase=138000  Vref=1  Vangle=0  VLF=1  angleLF=0
      settings: AttributesFormatString=|
      | %<ID>
      | %<Vbase>V
      | %<VLF>pu
      | %<angleLF>deg.
      | %<Name>
  bus39 : powerlib/Measurements/Load Flow Bus  LConnTagsString=a  ID=bus39  Vbase=138000  Vref=1  Vangle=0  VLF=1  angleLF=0
      settings: AttributesFormatString=|
      | %<ID>
      | %<Vbase>V
      | %<VLF>pu
      | %<angleLF>deg.
      | %<Name>
  bus390 : powerlib/Measurements/Load Flow Bus  LConnTagsString=a  ID=bus390  Vbase=138000  Vref=1  Vangle=0  VLF=1  angleLF=0
      settings: AttributesFormatString=|
      | %<ID>
      | %<Vbase>V
      | %<VLF>pu
      | %<angleLF>deg.
      | %<Name>
  bus391 : powerlib/Measurements/Load Flow Bus  LConnTagsString=a  ID=bus391  Vbase=138000  Vref=1  Vangle=0  VLF=1  angleLF=0
      settings: AttributesFormatString=|
      | %<ID>
      | %<Vbase>V
      | %<VLF>pu
      | %<angleLF>deg.
      | %<Name>
  bus392 : powerlib/Measurements/Load Flow Bus  LConnTagsString=a  ID=bus392  Vbase=138000  Vref=1  Vangle=0  VLF=1  angleLF=0
      settings: AttributesFormatString=|
      | %<ID>
      | %<Vbase>V
      | %<VLF>pu
      | %<angleLF>deg.
      | %<Name>
  bus393 : powerlib/Measurements/Load Flow Bus  LConnTagsString=a  ID=bus393  Vbase=138000  Vref=1  Vangle=0  VLF=1  angleLF=0
      settings: AttributesFormatString=|
      | %<ID>
      | %<Vbase>V
      | %<VLF>pu
      | %<angleLF>deg.
      | %<Name>
  bus394 : powerlib/Measurements/Load Flow Bus  LConnTagsString=a  ID=bus394  Vbase=138000  Vref=1  Vangle=0  VLF=1  angleLF=0
      settings: AttributesFormatString=|
      | %<ID>
      | %<Vbase>V
      | %<VLF>pu
      | %<angleLF>deg.
      | %<Name>
  bus395 : powerlib/Measurements/Load Flow Bus  LConnTagsString=a  ID=bus395  Vbase=138000  Vref=1  Vangle=0  VLF=1  angleLF=0
      settings: AttributesFormatString=|
      | %<ID>
      | %<Vbase>V
      | %<VLF>pu
      | %<angleLF>deg.
      | %<Name>
  bus396 : powerlib/Measurements/Load Flow Bus  LConnTagsString=a  ID=bus396  Vbase=138000  Vref=1  Vangle=0  VLF=1  angleLF=0
      settings: AttributesFormatString=|
      | %<ID>
      | %<Vbase>V
      | %<VLF>pu
      | %<angleLF>deg.
      | %<Name>
  bus397 : powerlib/Measurements/Load Flow Bus  LConnTagsString=a  ID=bus397  Vbase=138000  Vref=1  Vangle=0  VLF=1  angleLF=0
      settings: AttributesFormatString=|
      | %<ID>
      | %<Vbase>V
      | %<VLF>pu
      | %<angleLF>deg.
      | %<Name>
  bus398 : powerlib/Measurements/Load Flow Bus  LConnTagsString=a  ID=bus398  Vbase=138000  Vref=1  Vangle=0  VLF=1  angleLF=0
      settings: AttributesFormatString=|
      | %<ID>
      | %<Vbase>V
      | %<VLF>pu
      | %<angleLF>deg.
      | %<Name>
  bus399 : powerlib/Measurements/Load Flow Bus  LConnTagsString=a  ID=bus399  Vbase=138000  Vref=1  Vangle=0  VLF=1  angleLF=0
      settings: AttributesFormatString=|
      | %<ID>
      | %<Vbase>V
      | %<VLF>pu
      | %<angleLF>deg.
      | %<Name>
  bus4 : powerlib/Measurements/Load Flow Bus  LConnTagsString=a  ID=bus4  Vbase=138000  Vref=1  Vangle=0  VLF=1  angleLF=0
      settings: AttributesFormatString=|
      | %<ID>
      | %<Vbase>V
      | %<VLF>pu
      | %<angleLF>deg.
      | %<Name>
  bus40 : powerlib/Measurements/Load Flow Bus  LConnTagsString=a  ID=bus40  Vbase=138000  Vref=1  Vangle=0  VLF=1  angleLF=0
      settings: AttributesFormatString=|
      | %<ID>
      | %<Vbase>V
      | %<VLF>pu
      | %<angleLF>deg.
      | %<Name>
  bus400 : powerlib/Measurements/Load Flow Bus  LConnTagsString=a  ID=bus400  Vbase=138000  Vref=1  Vangle=0  VLF=1  angleLF=0
      settings: AttributesFormatString=|
      | %<ID>
      | %<Vbase>V
      | %<VLF>pu
      | %<angleLF>deg.
      | %<Name>
  bus401 : powerlib/Measurements/Load Flow Bus  LConnTagsString=a  ID=bus401  Vbase=138000  Vref=1  Vangle=0  VLF=1  angleLF=0
      settings: AttributesFormatString=|
      | %<ID>
      | %<Vbase>V
      | %<VLF>pu
      | %<angleLF>deg.
      | %<Name>
  bus402 : powerlib/Measurements/Load Flow Bus  LConnTagsString=a  ID=bus402  Vbase=138000  Vref=1  Vangle=0  VLF=1  angleLF=0
      settings: AttributesFormatString=|
      | %<ID>
      | %<Vbase>V
      | %<VLF>pu
      | %<angleLF>deg.
      | %<Name>
  bus403 : powerlib/Measurements/Load Flow Bus  LConnTagsString=a  ID=bus403  Vbase=138000  Vref=1  Vangle=0  VLF=1  angleLF=0
      settings: AttributesFormatString=|
      | %<ID>
      | %<Vbase>V
      | %<VLF>pu
      | %<angleLF>deg.
      | %<Name>
  bus404 : powerlib/Measurements/Load Flow Bus  LConnTagsString=a  ID=bus404  Vbase=138000  Vref=1  Vangle=0  VLF=1  angleLF=0
      settings: AttributesFormatString=|
      | %<ID>
      | %<Vbase>V
      | %<VLF>pu
      | %<angleLF>deg.
      | %<Name>
  bus405 : powerlib/Measurements/Load Flow Bus  LConnTagsString=a  ID=bus405  Vbase=138000  Vref=1  Vangle=0  VLF=1  angleLF=0
      settings: AttributesFormatString=|
      | %<ID>
      | %<Vbase>V
      | %<VLF>pu
      | %<angleLF>deg.
      | %<Name>
  bus406 : powerlib/Measurements/Load Flow Bus  LConnTagsString=a  ID=bus406  Vbase=138000  Vref=1  Vangle=0  VLF=1  angleLF=0
      settings: AttributesFormatString=|
      | %<ID>
      | %<Vbase>V
      | %<VLF>pu
      | %<angleLF>deg.
      | %<Name>
  bus407 : powerlib/Measurements/Load Flow Bus  LConnTagsString=a  ID=bus407  Vbase=138000  Vref=1  Vangle=0  VLF=1  angleLF=0
      settings: AttributesFormatString=|
      | %<ID>
      | %<Vbase>V
      | %<VLF>pu
      | %<angleLF>deg.
      | %<Name>
  bus408 : powerlib/Measurements/Load Flow Bus  LConnTagsString=a  ID=bus408  Vbase=138000  Vref=1  Vangle=0  VLF=1  angleLF=0
      settings: AttributesFormatString=|
      | %<ID>
      | %<Vbase>V
      | %<VLF>pu
      | %<angleLF>deg.
      | %<Name>
  bus409 : powerlib/Measurements/Load Flow Bus  LConnTagsString=a  ID=bus409  Vbase=138000  Vref=1  Vangle=0  VLF=1  angleLF=0
      settings: AttributesFormatString=|
      | %<ID>
      | %<Vbase>V
      | %<VLF>pu
      | %<angleLF>deg.
      | %<Name>
  bus41 : powerlib/Measurements/Load Flow Bus  LConnTagsString=a  ID=bus41  Vbase=138000  Vref=1  Vangle=0  VLF=1  angleLF=0
      settings: AttributesFormatString=|
      | %<ID>
      | %<Vbase>V
      | %<VLF>pu
      | %<angleLF>deg.
      | %<Name>
  bus410 : powerlib/Measurements/Load Flow Bus  LConnTagsString=a  ID=bus410  Vbase=138000  Vref=1  Vangle=0  VLF=1  angleLF=0
      settings: AttributesFormatString=|
      | %<ID>
      | %<Vbase>V
      | %<VLF>pu
      | %<angleLF>deg.
      | %<Name>
  bus411 : powerlib/Measurements/Load Flow Bus  LConnTagsString=a  ID=bus411  Vbase=138000  Vref=1  Vangle=0  VLF=1  angleLF=0
      settings: AttributesFormatString=|
      | %<ID>
      | %<Vbase>V
      | %<VLF>pu
      | %<angleLF>deg.
      | %<Name>
  bus412 : powerlib/Measurements/Load Flow Bus  LConnTagsString=a  ID=bus412  Vbase=138000  Vref=1  Vangle=0  VLF=1  angleLF=0
      settings: AttributesFormatString=|
      | %<ID>
      | %<Vbase>V
      | %<VLF>pu
      | %<angleLF>deg.
      | %<Name>
  bus413 : powerlib/Measurements/Load Flow Bus  LConnTagsString=a  ID=bus413  Vbase=138000  Vref=1  Vangle=0  VLF=1  angleLF=0
      settings: AttributesFormatString=|
      | %<ID>
      | %<Vbase>V
      | %<VLF>pu
      | %<angleLF>deg.
      | %<Name>
  bus414 : powerlib/Measurements/Load Flow Bus  LConnTagsString=a  ID=bus414  Vbase=138000  Vref=1  Vangle=0  VLF=1  angleLF=0
      settings: AttributesFormatString=|
      | %<ID>
      | %<Vbase>V
      | %<VLF>pu
      | %<angleLF>deg.
      | %<Name>
  bus415 : powerlib/Measurements/Load Flow Bus  LConnTagsString=a  ID=bus415  Vbase=138000  Vref=1  Vangle=0  VLF=1  angleLF=0
      settings: AttributesFormatString=|
      | %<ID>
      | %<Vbase>V
      | %<VLF>pu
      | %<angleLF>deg.
      | %<Name>
  bus416 : powerlib/Measurements/Load Flow Bus  LConnTagsString=a  ID=bus416  Vbase=138000  Vref=1  Vangle=0  VLF=1  angleLF=0
      settings: AttributesFormatString=|
      | %<ID>
      | %<Vbase>V
      | %<VLF>pu
      | %<angleLF>deg.
      | %<Name>
  bus417 : powerlib/Measurements/Load Flow Bus  LConnTagsString=a  ID=bus417  Vbase=138000  Vref=1  Vangle=0  VLF=1  angleLF=0
      settings: AttributesFormatString=|
      | %<ID>
      | %<Vbase>V
      | %<VLF>pu
      | %<angleLF>deg.
      | %<Name>
  bus418 : powerlib/Measurements/Load Flow Bus  LConnTagsString=a  ID=bus418  Vbase=138000  Vref=1  Vangle=0  VLF=1  angleLF=0
      settings: AttributesFormatString=|
      | %<ID>
      | %<Vbase>V
      | %<VLF>pu
      | %<angleLF>deg.
      | %<Name>
  bus419 : powerlib/Measurements/Load Flow Bus  LConnTagsString=a  ID=bus419  Vbase=230000  Vref=1  Vangle=0  VLF=1  angleLF=0
      settings: AttributesFormatString=|
      | %<ID>
      | %<Vbase>V
      | %<VLF>pu
      | %<angleLF>deg.
      | %<Name>
  bus42 : powerlib/Measurements/Load Flow Bus  LConnTagsString=a  ID=bus42  Vbase=138000  Vref=1  Vangle=0  VLF=1  angleLF=0
      settings: AttributesFormatString=|
      | %<ID>
      | %<Vbase>V
      | %<VLF>pu
      | %<angleLF>deg.
      | %<Name>
  bus420 : powerlib/Measurements/Load Flow Bus  LConnTagsString=a  ID=bus420  Vbase=230000  Vref=1  Vangle=0  VLF=1  angleLF=0
      settings: AttributesFormatString=|
      | %<ID>
      | %<Vbase>V
      | %<VLF>pu
      | %<angleLF>deg.
      | %<Name>
  bus421 : powerlib/Measurements/Load Flow Bus  LConnTagsString=a  ID=bus421  Vbase=230000  Vref=1  Vangle=0  VLF=1  angleLF=0
      settings: AttributesFormatString=|
      | %<ID>
      | %<Vbase>V
      | %<VLF>pu
      | %<angleLF>deg.
      | %<Name>
  bus422 : powerlib/Measurements/Load Flow Bus  LConnTagsString=a  ID=bus422  Vbase=230000  Vref=1  Vangle=0  VLF=1  angleLF=0
      settings: AttributesFormatString=|
      | %<ID>
      | %<Vbase>V
      | %<VLF>pu
      | %<angleLF>deg.
      | %<Name>
  bus423 : powerlib/Measurements/Load Flow Bus  LConnTagsString=a  ID=bus423  Vbase=230000  Vref=1  Vangle=0  VLF=1  angleLF=0
      settings: AttributesFormatString=|
      | %<ID>
      | %<Vbase>V
      | %<VLF>pu
      | %<angleLF>deg.
      | %<Name>
  bus424 : powerlib/Measurements/Load Flow Bus  LConnTagsString=a  ID=bus424  Vbase=230000  Vref=1  Vangle=0  VLF=1  angleLF=0
      settings: AttributesFormatString=|
      | %<ID>
      | %<Vbase>V
      | %<VLF>pu
      | %<angleLF>deg.
      | %<Name>
  bus425 : powerlib/Measurements/Load Flow Bus  LConnTagsString=a  ID=bus425  Vbase=230000  Vref=1  Vangle=0  VLF=1  angleLF=0
      settings: AttributesFormatString=|
      | %<ID>
      | %<Vbase>V
      | %<VLF>pu
      | %<angleLF>deg.
      | %<Name>
  bus426 : powerlib/Measurements/Load Flow Bus  LConnTagsString=a  ID=bus426  Vbase=230000  Vref=1  Vangle=0  VLF=1  angleLF=0
      settings: AttributesFormatString=|
      | %<ID>
      | %<Vbase>V
      | %<VLF>pu
      | %<angleLF>deg.
      | %<Name>
  bus427 : powerlib/Measurements/Load Flow Bus  LConnTagsString=a  ID=bus427  Vbase=230000  Vref=1  Vangle=0  VLF=1  angleLF=0
      settings: AttributesFormatString=|
      | %<ID>
      | %<Vbase>V
      | %<VLF>pu
      | %<angleLF>deg.
      | %<Name>
  bus428 : powerlib/Measurements/Load Flow Bus  LConnTagsString=a  ID=bus428  Vbase=230000  Vref=1  Vangle=0  VLF=1  angleLF=0
      settings: AttributesFormatString=|
      | %<ID>
      | %<Vbase>V
      | %<VLF>pu
      | %<angleLF>deg.
      | %<Name>
  bus429 : powerlib/Measurements/Load Flow Bus  LConnTagsString=a  ID=bus429  Vbase=230000  Vref=1  Vangle=0  VLF=1  angleLF=0
      settings: AttributesFormatString=|
      | %<ID>
      | %<Vbase>V
      | %<VLF>pu
      | %<angleLF>deg.
      | %<Name>
  bus43 : powerlib/Measurements/Load Flow Bus  LConnTagsString=a  ID=bus43  Vbase=138000  Vref=1  Vangle=0  VLF=1  angleLF=0
      settings: AttributesFormatString=|
      | %<ID>
      | %<Vbase>V
      | %<VLF>pu
      | %<angleLF>deg.
      | %<Name>
  bus430 : powerlib/Measurements/Load Flow Bus  LConnTagsString=a  ID=bus430  Vbase=230000  Vref=1  Vangle=0  VLF=1  angleLF=0
      settings: AttributesFormatString=|
      | %<ID>
      | %<Vbase>V
      | %<VLF>pu
      | %<angleLF>deg.
      | %<Name>
  bus431 : powerlib/Measurements/Load Flow Bus  LConnTagsString=a  ID=bus431  Vbase=230000  Vref=1  Vangle=0  VLF=1  angleLF=0
      settings: AttributesFormatString=|
      | %<ID>
      | %<Vbase>V
      | %<VLF>pu
      | %<angleLF>deg.
      | %<Name>
  bus432 : powerlib/Measurements/Load Flow Bus  LConnTagsString=a  ID=bus432  Vbase=230000  Vref=1  Vangle=0  VLF=1  angleLF=0
      settings: AttributesFormatString=|
      | %<ID>
      | %<Vbase>V
      | %<VLF>pu
      | %<angleLF>deg.
      | %<Name>
  bus433 : powerlib/Measurements/Load Flow Bus  LConnTagsString=a  ID=bus433  Vbase=230000  Vref=1  Vangle=0  VLF=1  angleLF=0
      settings: AttributesFormatString=|
      | %<ID>
      | %<Vbase>V
      | %<VLF>pu
      | %<angleLF>deg.
      | %<Name>
  bus434 : powerlib/Measurements/Load Flow Bus  LConnTagsString=a  ID=bus434  Vbase=230000  Vref=1  Vangle=0  VLF=1  angleLF=0
      settings: AttributesFormatString=|
      | %<ID>
      | %<Vbase>V
      | %<VLF>pu
      | %<angleLF>deg.
      | %<Name>
  bus435 : powerlib/Measurements/Load Flow Bus  LConnTagsString=a  ID=bus435  Vbase=230000  Vref=1  Vangle=0  VLF=1  angleLF=0
      settings: AttributesFormatString=|
      | %<ID>
      | %<Vbase>V
      | %<VLF>pu
      | %<angleLF>deg.
      | %<Name>
  bus436 : powerlib/Measurements/Load Flow Bus  LConnTagsString=a  ID=bus436  Vbase=230000  Vref=1  Vangle=0  VLF=1  angleLF=0
      settings: AttributesFormatString=|
      | %<ID>
      | %<Vbase>V
      | %<VLF>pu
      | %<angleLF>deg.
      | %<Name>
  bus437 : powerlib/Measurements/Load Flow Bus  LConnTagsString=a  ID=bus437  Vbase=230000  Vref=1  Vangle=0  VLF=1  angleLF=0
      settings: AttributesFormatString=|
      | %<ID>
      | %<Vbase>V
      | %<VLF>pu
      | %<angleLF>deg.
      | %<Name>
  bus438 : powerlib/Measurements/Load Flow Bus  LConnTagsString=a  ID=bus438  Vbase=230000  Vref=1  Vangle=0  VLF=1  angleLF=0
      settings: AttributesFormatString=|
      | %<ID>
      | %<Vbase>V
      | %<VLF>pu
      | %<angleLF>deg.
      | %<Name>
  bus439 : powerlib/Measurements/Load Flow Bus  LConnTagsString=a  ID=bus439  Vbase=230000  Vref=1  Vangle=0  VLF=1  angleLF=0
      settings: AttributesFormatString=|
      | %<ID>
      | %<Vbase>V
      | %<VLF>pu
      | %<angleLF>deg.
      | %<Name>
  bus44 : powerlib/Measurements/Load Flow Bus  LConnTagsString=a  ID=bus44  Vbase=138000  Vref=1  Vangle=0  VLF=1  angleLF=0
      settings: AttributesFormatString=|
      | %<ID>
      | %<Vbase>V
      | %<VLF>pu
      | %<angleLF>deg.
      | %<Name>
  bus440 : powerlib/Measurements/Load Flow Bus  LConnTagsString=a  ID=bus440  Vbase=230000  Vref=1  Vangle=0  VLF=1  angleLF=0
      settings: AttributesFormatString=|
      | %<ID>
      | %<Vbase>V
      | %<VLF>pu
      | %<angleLF>deg.
      | %<Name>
  bus441 : powerlib/Measurements/Load Flow Bus  LConnTagsString=a  ID=bus441  Vbase=230000  Vref=1  Vangle=0  VLF=1  angleLF=0
      settings: AttributesFormatString=|
      | %<ID>
      | %<Vbase>V
      | %<VLF>pu
      | %<angleLF>deg.
      | %<Name>
  bus442 : powerlib/Measurements/Load Flow Bus  LConnTagsString=a  ID=bus442  Vbase=230000  Vref=1  Vangle=0  VLF=1  angleLF=0
      settings: AttributesFormatString=|
      | %<ID>
      | %<Vbase>V
      | %<VLF>pu
      | %<angleLF>deg.
      | %<Name>
  bus443 : powerlib/Measurements/Load Flow Bus  LConnTagsString=a  ID=bus443  Vbase=230000  Vref=1  Vangle=0  VLF=1  angleLF=0
      settings: AttributesFormatString=|
      | %<ID>
      | %<Vbase>V
      | %<VLF>pu
      | %<angleLF>deg.
      | %<Name>
  bus444 : powerlib/Measurements/Load Flow Bus  LConnTagsString=a  ID=bus444  Vbase=230000  Vref=1  Vangle=0  VLF=1  angleLF=0
      settings: AttributesFormatString=|
      | %<ID>
      | %<Vbase>V
      | %<VLF>pu
      | %<angleLF>deg.
      | %<Name>
  bus445 : powerlib/Measurements/Load Flow Bus  LConnTagsString=a  ID=bus445  Vbase=230000  Vref=1  Vangle=0  VLF=1  angleLF=0
      settings: AttributesFormatString=|
      | %<ID>
      | %<Vbase>V
      | %<VLF>pu
      | %<angleLF>deg.
      | %<Name>
  bus446 : powerlib/Measurements/Load Flow Bus  LConnTagsString=a  ID=bus446  Vbase=230000  Vref=1  Vangle=0  VLF=1  angleLF=0
      settings: AttributesFormatString=|
      | %<ID>
      | %<Vbase>V
      | %<VLF>pu
      | %<angleLF>deg.
      | %<Name>
  bus447 : powerlib/Measurements/Load Flow Bus  LConnTagsString=a  ID=bus447  Vbase=230000  Vref=1  Vangle=0  VLF=1  angleLF=0
      settings: AttributesFormatString=|
      | %<ID>
      | %<Vbase>V
      | %<VLF>pu
      | %<angleLF>deg.
      | %<Name>
  bus448 : powerlib/Measurements/Load Flow Bus  LConnTagsString=a  ID=bus448  Vbase=230000  Vref=1  Vangle=0  VLF=1  angleLF=0
      settings: AttributesFormatString=|
      | %<ID>
      | %<Vbase>V
      | %<VLF>pu
      | %<angleLF>deg.
      | %<Name>
  bus449 : powerlib/Measurements/Load Flow Bus  LConnTagsString=a  ID=bus449  Vbase=230000  Vref=1  Vangle=0  VLF=1  angleLF=0
      settings: AttributesFormatString=|
      | %<ID>
      | %<Vbase>V
      | %<VLF>pu
      | %<angleLF>deg.
      | %<Name>
  bus45 : powerlib/Measurements/Load Flow Bus  LConnTagsString=a  ID=bus45  Vbase=138000  Vref=1  Vangle=0  VLF=1  angleLF=0
      settings: AttributesFormatString=|
      | %<ID>
      | %<Vbase>V
      | %<VLF>pu
      | %<angleLF>deg.
      | %<Name>
  bus450 : powerlib/Measurements/Load Flow Bus  LConnTagsString=a  ID=bus450  Vbase=230000  Vref=1  Vangle=0  VLF=1  angleLF=0
      settings: AttributesFormatString=|
      | %<ID>
      | %<Vbase>V
      | %<VLF>pu
      | %<angleLF>deg.
      | %<Name>
  bus451 : powerlib/Measurements/Load Flow Bus  LConnTagsString=a  ID=bus451  Vbase=230000  Vref=1  Vangle=0  VLF=1  angleLF=0
      settings: AttributesFormatString=|
      | %<ID>
      | %<Vbase>V
      | %<VLF>pu
      | %<angleLF>deg.
      | %<Name>
  bus452 : powerlib/Measurements/Load Flow Bus  LConnTagsString=a  ID=bus452  Vbase=230000  Vref=1  Vangle=0  VLF=1  angleLF=0
      settings: AttributesFormatString=|
      | %<ID>
      | %<Vbase>V
      | %<VLF>pu
      | %<angleLF>deg.
      | %<Name>
  bus453 : powerlib/Measurements/Load Flow Bus  LConnTagsString=a  ID=bus453  Vbase=230000  Vref=1  Vangle=0  VLF=1  angleLF=0
      settings: AttributesFormatString=|
      | %<ID>
      | %<Vbase>V
      | %<VLF>pu
      | %<angleLF>deg.
      | %<Name>
  bus454 : powerlib/Measurements/Load Flow Bus  LConnTagsString=a  ID=bus454  Vbase=230000  Vref=1  Vangle=0  VLF=1  angleLF=0
      settings: AttributesFormatString=|
      | %<ID>
      | %<Vbase>V
      | %<VLF>pu
      | %<angleLF>deg.
      | %<Name>
  bus455 : powerlib/Measurements/Load Flow Bus  LConnTagsString=a  ID=bus455  Vbase=230000  Vref=1  Vangle=0  VLF=1  angleLF=0
      settings: AttributesFormatString=|
      | %<ID>
      | %<Vbase>V
      | %<VLF>pu
      | %<angleLF>deg.
      | %<Name>
  bus456 : powerlib/Measurements/Load Flow Bus  LConnTagsString=a  ID=bus456  Vbase=230000  Vref=1  Vangle=0  VLF=1  angleLF=0
      settings: AttributesFormatString=|
      | %<ID>
      | %<Vbase>V
      | %<VLF>pu
      | %<angleLF>deg.
      | %<Name>
  bus457 : powerlib/Measurements/Load Flow Bus  LConnTagsString=a  ID=bus457  Vbase=230000  Vref=1  Vangle=0  VLF=1  angleLF=0
      settings: AttributesFormatString=|
      | %<ID>
      | %<Vbase>V
      | %<VLF>pu
      | %<angleLF>deg.
      | %<Name>
  bus458 : powerlib/Measurements/Load Flow Bus  LConnTagsString=a  ID=bus458  Vbase=230000  Vref=1  Vangle=0  VLF=1  angleLF=0
      settings: AttributesFormatString=|
      | %<ID>
      | %<Vbase>V
      | %<VLF>pu
      | %<angleLF>deg.
      | %<Name>
  bus459 : powerlib/Measurements/Load Flow Bus  LConnTagsString=a  ID=bus459  Vbase=230000  Vref=1  Vangle=0  VLF=1  angleLF=0
      settings: AttributesFormatString=|
      | %<ID>
      | %<Vbase>V
      | %<VLF>pu
      | %<angleLF>deg.
      | %<Name>
  bus46 : powerlib/Measurements/Load Flow Bus  LConnTagsString=a  ID=bus46  Vbase=138000  Vref=1  Vangle=0  VLF=1  angleLF=0
      settings: AttributesFormatString=|
      | %<ID>
      | %<Vbase>V
      | %<VLF>pu
      | %<angleLF>deg.
      | %<Name>
  bus460 : powerlib/Measurements/Load Flow Bus  LConnTagsString=a  ID=bus460  Vbase=230000  Vref=1  Vangle=0  VLF=1  angleLF=0
      settings: AttributesFormatString=|
      | %<ID>
      | %<Vbase>V
      | %<VLF>pu
      | %<angleLF>deg.
      | %<Name>
  bus461 : powerlib/Measurements/Load Flow Bus  LConnTagsString=a  ID=bus461  Vbase=230000  Vref=1  Vangle=0  VLF=1  angleLF=0
      settings: AttributesFormatString=|
      | %<ID>
      | %<Vbase>V
      | %<VLF>pu
      | %<angleLF>deg.
      | %<Name>
  bus462 : powerlib/Measurements/Load Flow Bus  LConnTagsString=a  ID=bus462  Vbase=230000  Vref=1  Vangle=0  VLF=1  angleLF=0
      settings: AttributesFormatString=|
      | %<ID>
      | %<Vbase>V
      | %<VLF>pu
      | %<angleLF>deg.
      | %<Name>
  bus463 : powerlib/Measurements/Load Flow Bus  LConnTagsString=a  ID=bus463  Vbase=230000  Vref=1  Vangle=0  VLF=1  angleLF=0
      settings: AttributesFormatString=|
      | %<ID>
      | %<Vbase>V
      | %<VLF>pu
      | %<angleLF>deg.
      | %<Name>
  bus464 : powerlib/Measurements/Load Flow Bus  LConnTagsString=a  ID=bus464  Vbase=230000  Vref=1  Vangle=0  VLF=1  angleLF=0
      settings: AttributesFormatString=|
      | %<ID>
      | %<Vbase>V
      | %<VLF>pu
      | %<angleLF>deg.
      | %<Name>
  bus465 : powerlib/Measurements/Load Flow Bus  LConnTagsString=a  ID=bus465  Vbase=230000  Vref=1  Vangle=0  VLF=1  angleLF=0
      settings: AttributesFormatString=|
      | %<ID>
      | %<Vbase>V
      | %<VLF>pu
      | %<angleLF>deg.
      | %<Name>
  bus466 : powerlib/Measurements/Load Flow Bus  LConnTagsString=a  ID=bus466  Vbase=230000  Vref=1  Vangle=0  VLF=1  angleLF=0
      settings: AttributesFormatString=|
      | %<ID>
      | %<Vbase>V
      | %<VLF>pu
      | %<angleLF>deg.
      | %<Name>
  bus467 : powerlib/Measurements/Load Flow Bus  LConnTagsString=a  ID=bus467  Vbase=230000  Vref=1  Vangle=0  VLF=1  angleLF=0
      settings: AttributesFormatString=|
      | %<ID>
      | %<Vbase>V
      | %<VLF>pu
      | %<angleLF>deg.
      | %<Name>
  bus468 : powerlib/Measurements/Load Flow Bus  LConnTagsString=a  ID=bus468  Vbase=230000  Vref=1  Vangle=0  VLF=1  angleLF=0
      settings: AttributesFormatString=|
      | %<ID>
      | %<Vbase>V
      | %<VLF>pu
      | %<angleLF>deg.
      | %<Name>
  bus469 : powerlib/Measurements/Load Flow Bus  LConnTagsString=a  ID=bus469  Vbase=230000  Vref=1  Vangle=0  VLF=1  angleLF=0
      settings: AttributesFormatString=|
      | %<ID>
      | %<Vbase>V
      | %<VLF>pu
      | %<angleLF>deg.
      | %<Name>
  bus47 : powerlib/Measurements/Load Flow Bus  LConnTagsString=a  ID=bus47  Vbase=138000  Vref=1  Vangle=0  VLF=1  angleLF=0
      settings: AttributesFormatString=|
      | %<ID>
      | %<Vbase>V
      | %<VLF>pu
      | %<angleLF>deg.
      | %<Name>
  bus470 : powerlib/Measurements/Load Flow Bus  LConnTagsString=a  ID=bus470  Vbase=230000  Vref=1  Vangle=0  VLF=1  angleLF=0
      settings: AttributesFormatString=|
      | %<ID>
      | %<Vbase>V
      | %<VLF>pu
      | %<angleLF>deg.
      | %<Name>
  bus471 : powerlib/Measurements/Load Flow Bus  LConnTagsString=a  ID=bus471  Vbase=230000  Vref=1  Vangle=0  VLF=1  angleLF=0
      settings: AttributesFormatString=|
      | %<ID>
      | %<Vbase>V
      | %<VLF>pu
      | %<angleLF>deg.
      | %<Name>
  bus472 : powerlib/Measurements/Load Flow Bus  LConnTagsString=a  ID=bus472  Vbase=230000  Vref=1  Vangle=0  VLF=1  angleLF=0
      settings: AttributesFormatString=|
      | %<ID>
      | %<Vbase>V
      | %<VLF>pu
      | %<angleLF>deg.
      | %<Name>
  bus473 : powerlib/Measurements/Load Flow Bus  LConnTagsString=a  ID=bus473  Vbase=230000  Vref=1  Vangle=0  VLF=1  angleLF=0
      settings: AttributesFormatString=|
      | %<ID>
      | %<Vbase>V
      | %<VLF>pu
      | %<angleLF>deg.
      | %<Name>
  bus474 : powerlib/Measurements/Load Flow Bus  LConnTagsString=a  ID=bus474  Vbase=230000  Vref=1  Vangle=0  VLF=1  angleLF=0
      settings: AttributesFormatString=|
      | %<ID>
      | %<Vbase>V
      | %<VLF>pu
      | %<angleLF>deg.
      | %<Name>
  bus475 : powerlib/Measurements/Load Flow Bus  LConnTagsString=a  ID=bus475  Vbase=230000  Vref=1  Vangle=0  VLF=1  angleLF=0
      settings: AttributesFormatString=|
      | %<ID>
      | %<Vbase>V
      | %<VLF>pu
      | %<angleLF>deg.
      | %<Name>
  bus476 : powerlib/Measurements/Load Flow Bus  LConnTagsString=a  ID=bus476  Vbase=230000  Vref=1  Vangle=0  VLF=1  angleLF=0
      settings: AttributesFormatString=|
      | %<ID>
      | %<Vbase>V
      | %<VLF>pu
      | %<angleLF>deg.
      | %<Name>
  bus477 : powerlib/Measurements/Load Flow Bus  LConnTagsString=a  ID=bus477  Vbase=230000  Vref=1  Vangle=0  VLF=1  angleLF=0
      settings: AttributesFormatString=|
      | %<ID>
      | %<Vbase>V
      | %<VLF>pu
      | %<angleLF>deg.
      | %<Name>
  bus478 : powerlib/Measurements/Load Flow Bus  LConnTagsString=a  ID=bus478  Vbase=230000  Vref=1  Vangle=0  VLF=1  angleLF=0
      settings: AttributesFormatString=|
      | %<ID>
      | %<Vbase>V
      | %<VLF>pu
      | %<angleLF>deg.
      | %<Name>
  bus479 : powerlib/Measurements/Load Flow Bus  LConnTagsString=a  ID=bus479  Vbase=230000  Vref=1  Vangle=0  VLF=1  angleLF=0
      settings: AttributesFormatString=|
      | %<ID>
      | %<Vbase>V
      | %<VLF>pu
      | %<angleLF>deg.
      | %<Name>
  bus48 : powerlib/Measurements/Load Flow Bus  LConnTagsString=a  ID=bus48  Vbase=138000  Vref=1  Vangle=0  VLF=1  angleLF=0
      settings: AttributesFormatString=|
      | %<ID>
      | %<Vbase>V
      | %<VLF>pu
      | %<angleLF>deg.
      | %<Name>
  bus480 : powerlib/Measurements/Load Flow Bus  LConnTagsString=a  ID=bus480  Vbase=230000  Vref=1  Vangle=0  VLF=1  angleLF=0
      settings: AttributesFormatString=|
      | %<ID>
      | %<Vbase>V
      | %<VLF>pu
      | %<angleLF>deg.
      | %<Name>
  bus481 : powerlib/Measurements/Load Flow Bus  LConnTagsString=a  ID=bus481  Vbase=230000  Vref=1  Vangle=0  VLF=1  angleLF=0
      settings: AttributesFormatString=|
      | %<ID>
      | %<Vbase>V
      | %<VLF>pu
      | %<angleLF>deg.
      | %<Name>
  bus482 : powerlib/Measurements/Load Flow Bus  LConnTagsString=a  ID=bus482  Vbase=230000  Vref=1  Vangle=0  VLF=1  angleLF=0
      settings: AttributesFormatString=|
      | %<ID>
      | %<Vbase>V
      | %<VLF>pu
      | %<angleLF>deg.
      | %<Name>
  bus483 : powerlib/Measurements/Load Flow Bus  LConnTagsString=a  ID=bus483  Vbase=230000  Vref=1  Vangle=0  VLF=1  angleLF=0
      settings: AttributesFormatString=|
      | %<ID>
      | %<Vbase>V
      | %<VLF>pu
      | %<angleLF>deg.
      | %<Name>
  bus484 : powerlib/Measurements/Load Flow Bus  LConnTagsString=a  ID=bus484  Vbase=230000  Vref=1  Vangle=0  VLF=1  angleLF=0
      settings: AttributesFormatString=|
      | %<ID>
      | %<Vbase>V
      | %<VLF>pu
      | %<angleLF>deg.
      | %<Name>
  bus485 : powerlib/Measurements/Load Flow Bus  LConnTagsString=a  ID=bus485  Vbase=230000  Vref=1  Vangle=0  VLF=1  angleLF=0
      settings: AttributesFormatString=|
      | %<ID>
      | %<Vbase>V
      | %<VLF>pu
      | %<angleLF>deg.
      | %<Name>
  bus486 : powerlib/Measurements/Load Flow Bus  LConnTagsString=a  ID=bus486  Vbase=230000  Vref=1  Vangle=0  VLF=1  angleLF=0
      settings: AttributesFormatString=|
      | %<ID>
      | %<Vbase>V
      | %<VLF>pu
      | %<angleLF>deg.
      | %<Name>
  bus487 : powerlib/Measurements/Load Flow Bus  LConnTagsString=a  ID=bus487  Vbase=230000  Vref=1  Vangle=0  VLF=1  angleLF=0
      settings: AttributesFormatString=|
      | %<ID>
      | %<Vbase>V
      | %<VLF>pu
      | %<angleLF>deg.
      | %<Name>
  bus488 : powerlib/Measurements/Load Flow Bus  LConnTagsString=a  ID=bus488  Vbase=230000  Vref=1  Vangle=0  VLF=1  angleLF=0
      settings: AttributesFormatString=|
      | %<ID>
      | %<Vbase>V
      | %<VLF>pu
      | %<angleLF>deg.
      | %<Name>
  bus489 : powerlib/Measurements/Load Flow Bus  LConnTagsString=a  ID=bus489  Vbase=230000  Vref=1  Vangle=0  VLF=1  angleLF=0
      settings: AttributesFormatString=|
      | %<ID>
      | %<Vbase>V
      | %<VLF>pu
      | %<angleLF>deg.
      | %<Name>
  bus49 : powerlib/Measurements/Load Flow Bus  LConnTagsString=a  ID=bus49  Vbase=138000  Vref=1  Vangle=0  VLF=1  angleLF=0
      settings: AttributesFormatString=|
      | %<ID>
      | %<Vbase>V
      | %<VLF>pu
      | %<angleLF>deg.
      | %<Name>
  bus490 : powerlib/Measurements/Load Flow Bus  LConnTagsString=a  ID=bus490  Vbase=230000  Vref=1  Vangle=0  VLF=1  angleLF=0
      settings: AttributesFormatString=|
      | %<ID>
      | %<Vbase>V
      | %<VLF>pu
      | %<angleLF>deg.
      | %<Name>
  bus491 : powerlib/Measurements/Load Flow Bus  LConnTagsString=a  ID=bus491  Vbase=230000  Vref=1  Vangle=0  VLF=1  angleLF=0
      settings: AttributesFormatString=|
      | %<ID>
      | %<Vbase>V
      | %<VLF>pu
      | %<angleLF>deg.
      | %<Name>
  bus492 : powerlib/Measurements/Load Flow Bus  LConnTagsString=a  ID=bus492  Vbase=230000  Vref=1  Vangle=0  VLF=1  angleLF=0
      settings: AttributesFormatString=|
      | %<ID>
      | %<Vbase>V
      | %<VLF>pu
      | %<angleLF>deg.
      | %<Name>
  bus493 : powerlib/Measurements/Load Flow Bus  LConnTagsString=a  ID=bus493  Vbase=345000  Vref=1  Vangle=0  VLF=1  angleLF=0
      settings: AttributesFormatString=|
      | %<ID>
      | %<Vbase>V
      | %<VLF>pu
      | %<angleLF>deg.
      | %<Name>
  bus494 : powerlib/Measurements/Load Flow Bus  LConnTagsString=a  ID=bus494  Vbase=345000  Vref=1  Vangle=0  VLF=1  angleLF=0
      settings: AttributesFormatString=|
      | %<ID>
      | %<Vbase>V
      | %<VLF>pu
      | %<angleLF>deg.
      | %<Name>
  bus495 : powerlib/Measurements/Load Flow Bus  LConnTagsString=a  ID=bus495  Vbase=345000  Vref=1  Vangle=0  VLF=1  angleLF=0
      settings: AttributesFormatString=|
      | %<ID>
      | %<Vbase>V
      | %<VLF>pu
      | %<angleLF>deg.
      | %<Name>
  bus496 : powerlib/Measurements/Load Flow Bus  LConnTagsString=a  ID=bus496  Vbase=345000  Vref=1  Vangle=0  VLF=1  angleLF=0
      settings: AttributesFormatString=|
      | %<ID>
      | %<Vbase>V
      | %<VLF>pu
      | %<angleLF>deg.
      | %<Name>
  bus497 : powerlib/Measurements/Load Flow Bus  LConnTagsString=a  ID=bus497  Vbase=345000  Vref=1  Vangle=0  VLF=1  angleLF=0
      settings: AttributesFormatString=|
      | %<ID>
      | %<Vbase>V
      | %<VLF>pu
      | %<angleLF>deg.
      | %<Name>
  bus498 : powerlib/Measurements/Load Flow Bus  LConnTagsString=a  ID=bus498  Vbase=345000  Vref=1  Vangle=0  VLF=1  angleLF=0
      settings: AttributesFormatString=|
      | %<ID>
      | %<Vbase>V
      | %<VLF>pu
      | %<angleLF>deg.
      | %<Name>
  bus499 : powerlib/Measurements/Load Flow Bus  LConnTagsString=a  ID=bus499  Vbase=345000  Vref=1  Vangle=0  VLF=1  angleLF=0
      settings: AttributesFormatString=|
      | %<ID>
      | %<Vbase>V
      | %<VLF>pu
      | %<angleLF>deg.
      | %<Name>
  bus5 : powerlib/Measurements/Load Flow Bus  LConnTagsString=a  ID=bus5  Vbase=138000  Vref=1  Vangle=0  VLF=1  angleLF=0
      settings: AttributesFormatString=|
      | %<ID>
      | %<Vbase>V
      | %<VLF>pu
      | %<angleLF>deg.
      | %<Name>
  bus50 : powerlib/Measurements/Load Flow Bus  LConnTagsString=a  ID=bus50  Vbase=138000  Vref=1  Vangle=0  VLF=1  angleLF=0
      settings: AttributesFormatString=|
      | %<ID>
      | %<Vbase>V
      | %<VLF>pu
      | %<angleLF>deg.
      | %<Name>
  bus500 : powerlib/Measurements/Load Flow Bus  LConnTagsString=a  ID=bus500  Vbase=345000  Vref=1  Vangle=0  VLF=1  angleLF=0
      settings: AttributesFormatString=|
      | %<ID>
      | %<Vbase>V
      | %<VLF>pu
      | %<angleLF>deg.
      | %<Name>
  bus501 : powerlib/Measurements/Load Flow Bus  LConnTagsString=a  ID=bus501  Vbase=345000  Vref=1  Vangle=0  VLF=1  angleLF=0
      settings: AttributesFormatString=|
      | %<ID>
      | %<Vbase>V
      | %<VLF>pu
      | %<angleLF>deg.
      | %<Name>
  bus502 : powerlib/Measurements/Load Flow Bus  LConnTagsString=a  ID=bus502  Vbase=345000  Vref=1  Vangle=0  VLF=1  angleLF=0
      settings: AttributesFormatString=|
      | %<ID>
      | %<Vbase>V
      | %<VLF>pu
      | %<angleLF>deg.
      | %<Name>
  bus503 : powerlib/Measurements/Load Flow Bus  LConnTagsString=a  ID=bus503  Vbase=345000  Vref=1  Vangle=0  VLF=1  angleLF=0
      settings: AttributesFormatString=|
      | %<ID>
      | %<Vbase>V
      | %<VLF>pu
      | %<angleLF>deg.
      | %<Name>
  bus504 : powerlib/Measurements/Load Flow Bus  LConnTagsString=a  ID=bus504  Vbase=345000  Vref=1  Vangle=0  VLF=1  angleLF=0
      settings: AttributesFormatString=|
      | %<ID>
      | %<Vbase>V
      | %<VLF>pu
      | %<angleLF>deg.
      | %<Name>
  bus505 : powerlib/Measurements/Load Flow Bus  LConnTagsString=a  ID=bus505  Vbase=345000  Vref=1  Vangle=0  VLF=1  angleLF=0
      settings: AttributesFormatString=|
      | %<ID>
      | %<Vbase>V
      | %<VLF>pu
      | %<angleLF>deg.
      | %<Name>
  bus506 : powerlib/Measurements/Load Flow Bus  LConnTagsString=a  ID=bus506  Vbase=345000  Vref=1  Vangle=0  VLF=1  angleLF=0
      settings: AttributesFormatString=|
      | %<ID>
      | %<Vbase>V
      | %<VLF>pu
      | %<angleLF>deg.
      | %<Name>
  bus507 : powerlib/Measurements/Load Flow Bus  LConnTagsString=a  ID=bus507  Vbase=345000  Vref=1  Vangle=0  VLF=1  angleLF=0
      settings: AttributesFormatString=|
      | %<ID>
      | %<Vbase>V
      | %<VLF>pu
      | %<angleLF>deg.
      | %<Name>
  bus508 : powerlib/Measurements/Load Flow Bus  LConnTagsString=a  ID=bus508  Vbase=345000  Vref=1  Vangle=0  VLF=1  angleLF=0
      settings: AttributesFormatString=|
      | %<ID>
      | %<Vbase>V
      | %<VLF>pu
      | %<angleLF>deg.
      | %<Name>
  bus509 : powerlib/Measurements/Load Flow Bus  LConnTagsString=a  ID=bus509  Vbase=345000  Vref=1  Vangle=0  VLF=1  angleLF=0
      settings: AttributesFormatString=|
      | %<ID>
      | %<Vbase>V
      | %<VLF>pu
      | %<angleLF>deg.
      | %<Name>
  bus51 : powerlib/Measurements/Load Flow Bus  LConnTagsString=a  ID=bus51  Vbase=138000  Vref=1  Vangle=0  VLF=1  angleLF=0
      settings: AttributesFormatString=|
      | %<ID>
      | %<Vbase>V
      | %<VLF>pu
      | %<angleLF>deg.
      | %<Name>
  bus510 : powerlib/Measurements/Load Flow Bus  LConnTagsString=a  ID=bus510  Vbase=345000  Vref=1  Vangle=0  VLF=1  angleLF=0
      settings: AttributesFormatString=|
      | %<ID>
      | %<Vbase>V
      | %<VLF>pu
      | %<angleLF>deg.
      | %<Name>
  bus511 : powerlib/Measurements/Load Flow Bus  LConnTagsString=a  ID=bus511  Vbase=345000  Vref=1  Vangle=0  VLF=1  angleLF=0
      settings: AttributesFormatString=|
      | %<ID>
      | %<Vbase>V
      | %<VLF>pu
      | %<angleLF>deg.
      | %<Name>
  bus512 : powerlib/Measurements/Load Flow Bus  LConnTagsString=a  ID=bus512  Vbase=345000  Vref=1  Vangle=0  VLF=1  angleLF=0
      settings: AttributesFormatString=|
      | %<ID>
      | %<Vbase>V
      | %<VLF>pu
      | %<angleLF>deg.
      | %<Name>
  bus513 : powerlib/Measurements/Load Flow Bus  LConnTagsString=a  ID=bus513  Vbase=345000  Vref=1  Vangle=0  VLF=1  angleLF=0
      settings: AttributesFormatString=|
      | %<ID>
      | %<Vbase>V
      | %<VLF>pu
      | %<angleLF>deg.
      | %<Name>
  bus514 : powerlib/Measurements/Load Flow Bus  LConnTagsString=a  ID=bus514  Vbase=345000  Vref=1  Vangle=0  VLF=1  angleLF=0
      settings: AttributesFormatString=|
      | %<ID>
      | %<Vbase>V
      | %<VLF>pu
      | %<angleLF>deg.
      | %<Name>
  bus515 : powerlib/Measurements/Load Flow Bus  LConnTagsString=a  ID=bus515  Vbase=440000  Vref=1  Vangle=0  VLF=1  angleLF=0
      settings: AttributesFormatString=|
      | %<ID>
      | %<Vbase>V
      | %<VLF>pu
      | %<angleLF>deg.
      | %<Name>
  bus516 : powerlib/Measurements/Load Flow Bus  LConnTagsString=a  ID=bus516  Vbase=440000  Vref=1  Vangle=0  VLF=1  angleLF=0
      settings: AttributesFormatString=|
      | %<ID>
      | %<Vbase>V
      | %<VLF>pu
      | %<angleLF>deg.
      | %<Name>
  bus517 : powerlib/Measurements/Load Flow Bus  LConnTagsString=a  ID=bus517  Vbase=440000  Vref=1  Vangle=0  VLF=1  angleLF=0
      settings: AttributesFormatString=|
      | %<ID>
      | %<Vbase>V
      | %<VLF>pu
      | %<angleLF>deg.
      | %<Name>
  bus518 : powerlib/Measurements/Load Flow Bus  LConnTagsString=a  ID=bus518  Vbase=440000  Vref=1  Vangle=0  VLF=1  angleLF=0
      settings: AttributesFormatString=|
      | %<ID>
      | %<Vbase>V
      | %<VLF>pu
      | %<angleLF>deg.
      | %<Name>
  bus519 : powerlib/Measurements/Load Flow Bus  LConnTagsString=a  ID=bus519  Vbase=440000  Vref=1  Vangle=0  VLF=1  angleLF=0
      settings: AttributesFormatString=|
      | %<ID>
      | %<Vbase>V
      | %<VLF>pu
      | %<angleLF>deg.
      | %<Name>
  bus52 : powerlib/Measurements/Load Flow Bus  LConnTagsString=a  ID=bus52  Vbase=138000  Vref=1  Vangle=0  VLF=1  angleLF=0
      settings: AttributesFormatString=|
      | %<ID>
      | %<Vbase>V
      | %<VLF>pu
      | %<angleLF>deg.
      | %<Name>
  bus520 : powerlib/Measurements/Load Flow Bus  LConnTagsString=a  ID=bus520  Vbase=440000  Vref=1  Vangle=0  VLF=1  angleLF=0
      settings: AttributesFormatString=|
      | %<ID>
      | %<Vbase>V
      | %<VLF>pu
      | %<angleLF>deg.
      | %<Name>
  bus521 : powerlib/Measurements/Load Flow Bus  LConnTagsString=a  ID=bus521  Vbase=440000  Vref=1  Vangle=0  VLF=1  angleLF=0
      settings: AttributesFormatString=|
      | %<ID>
      | %<Vbase>V
      | %<VLF>pu
      | %<angleLF>deg.
      | %<Name>
  bus522 : powerlib/Measurements/Load Flow Bus  LConnTagsString=a  ID=bus522  Vbase=440000  Vref=1  Vangle=0  VLF=1  angleLF=0
      settings: AttributesFormatString=|
      | %<ID>
      | %<Vbase>V
      | %<VLF>pu
      | %<angleLF>deg.
      | %<Name>
  bus523 : powerlib/Measurements/Load Flow Bus  LConnTagsString=a  ID=bus523  Vbase=440000  Vref=1  Vangle=0  VLF=1  angleLF=0
      settings: AttributesFormatString=|
      | %<ID>
      | %<Vbase>V
      | %<VLF>pu
      | %<angleLF>deg.
      | %<Name>
  bus524 : powerlib/Measurements/Load Flow Bus  LConnTagsString=a  ID=bus524  Vbase=440000  Vref=1  Vangle=0  VLF=1  angleLF=0
      settings: AttributesFormatString=|
      | %<ID>
      | %<Vbase>V
      | %<VLF>pu
      | %<angleLF>deg.
      | %<Name>
  bus525 : powerlib/Measurements/Load Flow Bus  LConnTagsString=a  ID=bus525  Vbase=440000  Vref=1  Vangle=0  VLF=1  angleLF=0
      settings: AttributesFormatString=|
      | %<ID>
      | %<Vbase>V
      | %<VLF>pu
      | %<angleLF>deg.
      | %<Name>
  bus526 : powerlib/Measurements/Load Flow Bus  LConnTagsString=a  ID=bus526  Vbase=440000  Vref=1  Vangle=0  VLF=1  angleLF=0
      settings: AttributesFormatString=|
      | %<ID>
      | %<Vbase>V
      | %<VLF>pu
      | %<angleLF>deg.
      | %<Name>
  bus527 : powerlib/Measurements/Load Flow Bus  LConnTagsString=a  ID=bus527  Vbase=440000  Vref=1  Vangle=0  VLF=1  angleLF=0
      settings: AttributesFormatString=|
      | %<ID>
      | %<Vbase>V
      | %<VLF>pu
      | %<angleLF>deg.
      | %<Name>
  bus528 : powerlib/Measurements/Load Flow Bus  LConnTagsString=a  ID=bus528  Vbase=440000  Vref=1  Vangle=0  VLF=1  angleLF=0
      settings: AttributesFormatString=|
      | %<ID>
      | %<Vbase>V
      | %<VLF>pu
      | %<angleLF>deg.
      | %<Name>
  bus529 : powerlib/Measurements/Load Flow Bus  LConnTagsString=a  ID=bus529  Vbase=440000  Vref=1  Vangle=0  VLF=1  angleLF=0
      settings: AttributesFormatString=|
      | %<ID>
      | %<Vbase>V
      | %<VLF>pu
      | %<angleLF>deg.
      | %<Name>
  bus53 : powerlib/Measurements/Load Flow Bus  LConnTagsString=a  ID=bus53  Vbase=138000  Vref=1  Vangle=0  VLF=1  angleLF=0
      settings: AttributesFormatString=|
      | %<ID>
      | %<Vbase>V
      | %<VLF>pu
      | %<angleLF>deg.
      | %<Name>
  bus530 : powerlib/Measurements/Load Flow Bus  LConnTagsString=a  ID=bus530  Vbase=440000  Vref=1  Vangle=0  VLF=1  angleLF=0
      settings: AttributesFormatString=|
      | %<ID>
      | %<Vbase>V
      | %<VLF>pu
      | %<angleLF>deg.
      | %<Name>
  bus531 : powerlib/Measurements/Load Flow Bus  LConnTagsString=a  ID=bus531  Vbase=440000  Vref=1  Vangle=0  VLF=1  angleLF=0
      settings: AttributesFormatString=|
      | %<ID>
      | %<Vbase>V
      | %<VLF>pu
      | %<angleLF>deg.
      | %<Name>
  bus532 : powerlib/Measurements/Load Flow Bus  LConnTagsString=a  ID=bus532  Vbase=440000  Vref=1  Vangle=0  VLF=1  angleLF=0
      settings: AttributesFormatString=|
      | %<ID>
      | %<Vbase>V
      | %<VLF>pu
      | %<angleLF>deg.
      | %<Name>
  bus533 : powerlib/Measurements/Load Flow Bus  LConnTagsString=a  ID=bus533  Vbase=440000  Vref=1  Vangle=0  VLF=1  angleLF=0
      settings: AttributesFormatString=|
      | %<ID>
      | %<Vbase>V
      | %<VLF>pu
      | %<angleLF>deg.
      | %<Name>
  bus534 : powerlib/Measurements/Load Flow Bus  LConnTagsString=a  ID=bus534  Vbase=500000  Vref=1  Vangle=0  VLF=1  angleLF=0
      settings: AttributesFormatString=|
      | %<ID>
      | %<Vbase>V
      | %<VLF>pu
      | %<angleLF>deg.
      | %<Name>
  bus535 : powerlib/Measurements/Load Flow Bus  LConnTagsString=a  ID=bus535  Vbase=500000  Vref=1  Vangle=0  VLF=1  angleLF=0
      settings: AttributesFormatString=|
      | %<ID>
      | %<Vbase>V
      | %<VLF>pu
      | %<angleLF>deg.
      | %<Name>
  bus536 : powerlib/Measurements/Load Flow Bus  LConnTagsString=a  ID=bus536  Vbase=500000  Vref=1  Vangle=0  VLF=1  angleLF=0
      settings: AttributesFormatString=|
      | %<ID>
      | %<Vbase>V
      | %<VLF>pu
      | %<angleLF>deg.
      | %<Name>
  bus537 : powerlib/Measurements/Load Flow Bus  LConnTagsString=a  ID=bus537  Vbase=500000  Vref=1  Vangle=0  VLF=1  angleLF=0
      settings: AttributesFormatString=|
      | %<ID>
      | %<Vbase>V
      | %<VLF>pu
      | %<angleLF>deg.
      | %<Name>
  bus538 : powerlib/Measurements/Load Flow Bus  LConnTagsString=a  ID=bus538  Vbase=500000  Vref=1  Vangle=0  VLF=1  angleLF=0
      settings: AttributesFormatString=|
      | %<ID>
      | %<Vbase>V
      | %<VLF>pu
      | %<angleLF>deg.
      | %<Name>
  bus539 : powerlib/Measurements/Load Flow Bus  LConnTagsString=a  ID=bus539  Vbase=500000  Vref=1  Vangle=0  VLF=1  angleLF=0
      settings: AttributesFormatString=|
      | %<ID>
      | %<Vbase>V
      | %<VLF>pu
      | %<angleLF>deg.
      | %<Name>
  bus54 : powerlib/Measurements/Load Flow Bus  LConnTagsString=a  ID=bus54  Vbase=138000  Vref=1  Vangle=0  VLF=1  angleLF=0
      settings: AttributesFormatString=|
      | %<ID>
      | %<Vbase>V
      | %<VLF>pu
      | %<angleLF>deg.
      | %<Name>
  bus540 : powerlib/Measurements/Load Flow Bus  LConnTagsString=a  ID=bus540  Vbase=500000  Vref=1  Vangle=0  VLF=1  angleLF=0
      settings: AttributesFormatString=|
      | %<ID>
      | %<Vbase>V
      | %<VLF>pu
      | %<angleLF>deg.
      | %<Name>
  bus541 : powerlib/Measurements/Load Flow Bus  LConnTagsString=a  ID=bus541  Vbase=500000  Vref=1  Vangle=0  VLF=1  angleLF=0
      settings: AttributesFormatString=|
      | %<ID>
      | %<Vbase>V
      | %<VLF>pu
      | %<angleLF>deg.
      | %<Name>
  bus542 : powerlib/Measurements/Load Flow Bus  LConnTagsString=a  ID=bus542  Vbase=500000  Vref=1  Vangle=0  VLF=1  angleLF=0
      settings: AttributesFormatString=|
      | %<ID>
      | %<Vbase>V
      | %<VLF>pu
      | %<angleLF>deg.
      | %<Name>
  bus543 : powerlib/Measurements/Load Flow Bus  LConnTagsString=a  ID=bus543  Vbase=500000  Vref=1  Vangle=0  VLF=1  angleLF=0
      settings: AttributesFormatString=|
      | %<ID>
      | %<Vbase>V
      | %<VLF>pu
      | %<angleLF>deg.
      | %<Name>
  bus544 : powerlib/Measurements/Load Flow Bus  LConnTagsString=a  ID=bus544  Vbase=500000  Vref=1  Vangle=0  VLF=1  angleLF=0
      settings: AttributesFormatString=|
      | %<ID>
      | %<Vbase>V
      | %<VLF>pu
      | %<angleLF>deg.
      | %<Name>
  bus545 : powerlib/Measurements/Load Flow Bus  LConnTagsString=a  ID=bus545  Vbase=500000  Vref=1  Vangle=0  VLF=1  angleLF=0
      settings: AttributesFormatString=|
      | %<ID>
      | %<Vbase>V
      | %<VLF>pu
      | %<angleLF>deg.
      | %<Name>
  bus546 : powerlib/Measurements/Load Flow Bus  LConnTagsString=a  ID=bus546  Vbase=500000  Vref=1  Vangle=0  VLF=1  angleLF=0
      settings: AttributesFormatString=|
      | %<ID>
      | %<Vbase>V
      | %<VLF>pu
      | %<angleLF>deg.
      | %<Name>
  bus547 : powerlib/Measurements/Load Flow Bus  LConnTagsString=a  ID=bus547  Vbase=500000  Vref=1  Vangle=0  VLF=1  angleLF=0
      settings: AttributesFormatString=|
      | %<ID>
      | %<Vbase>V
      | %<VLF>pu
      | %<angleLF>deg.
      | %<Name>
  bus548 : powerlib/Measurements/Load Flow Bus  LConnTagsString=a  ID=bus548  Vbase=500000  Vref=1  Vangle=0  VLF=1  angleLF=0
      settings: AttributesFormatString=|
      | %<ID>
      | %<Vbase>V
      | %<VLF>pu
      | %<angleLF>deg.
      | %<Name>
  bus549 : powerlib/Measurements/Load Flow Bus  LConnTagsString=a  ID=bus549  Vbase=500000  Vref=1  Vangle=0  VLF=1  angleLF=0
      settings: AttributesFormatString=|
      | %<ID>
      | %<Vbase>V
      | %<VLF>pu
      | %<angleLF>deg.
      | %<Name>
  bus55 : powerlib/Measurements/Load Flow Bus  LConnTagsString=a  ID=bus55  Vbase=138000  Vref=1  Vangle=0  VLF=1  angleLF=0
      settings: AttributesFormatString=|
      | %<ID>
      | %<Vbase>V
      | %<VLF>pu
      | %<angleLF>deg.
      | %<Name>
  bus550 : powerlib/Measurements/Load Flow Bus  LConnTagsString=a  ID=bus550  Vbase=500000  Vref=1  Vangle=0  VLF=1  angleLF=0
      settings: AttributesFormatString=|
      | %<ID>
      | %<Vbase>V
      | %<VLF>pu
      | %<angleLF>deg.
      | %<Name>
  bus551 : powerlib/Measurements/Load Flow Bus  LConnTagsString=a  ID=bus551  Vbase=500000  Vref=1  Vangle=0  VLF=1  angleLF=0
      settings: AttributesFormatString=|
      | %<ID>
      | %<Vbase>V
      | %<VLF>pu
      | %<angleLF>deg.
      | %<Name>
  bus552 : powerlib/Measurements/Load Flow Bus  LConnTagsString=a  ID=bus552  Vbase=500000  Vref=1  Vangle=0  VLF=1  angleLF=0
      settings: AttributesFormatString=|
      | %<ID>
      | %<Vbase>V
      | %<VLF>pu
      | %<angleLF>deg.
      | %<Name>
  bus553 : powerlib/Measurements/Load Flow Bus  LConnTagsString=a  ID=bus553  Vbase=500000  Vref=1  Vangle=0  VLF=1  angleLF=0
      settings: AttributesFormatString=|
      | %<ID>
      | %<Vbase>V
      | %<VLF>pu
      | %<angleLF>deg.
      | %<Name>
  bus554 : powerlib/Measurements/Load Flow Bus  LConnTagsString=a  ID=bus554  Vbase=500000  Vref=1  Vangle=0  VLF=1  angleLF=0
      settings: AttributesFormatString=|
      | %<ID>
      | %<Vbase>V
      | %<VLF>pu
      | %<angleLF>deg.
      | %<Name>
  bus555 : powerlib/Measurements/Load Flow Bus  LConnTagsString=a  ID=bus555  Vbase=500000  Vref=1  Vangle=0  VLF=1  angleLF=0
      settings: AttributesFormatString=|
      | %<ID>
      | %<Vbase>V
      | %<VLF>pu
      | %<angleLF>deg.
      | %<Name>
  bus556 : powerlib/Measurements/Load Flow Bus  LConnTagsString=a  ID=bus556  Vbase=500000  Vref=1  Vangle=0  VLF=1  angleLF=0
      settings: AttributesFormatString=|
      | %<ID>
      | %<Vbase>V
      | %<VLF>pu
      | %<angleLF>deg.
      | %<Name>
  bus557 : powerlib/Measurements/Load Flow Bus  LConnTagsString=a  ID=bus557  Vbase=500000  Vref=1  Vangle=0  VLF=1  angleLF=0
      settings: AttributesFormatString=|
      | %<ID>
      | %<Vbase>V
      | %<VLF>pu
      | %<angleLF>deg.
      | %<Name>
  bus558 : powerlib/Measurements/Load Flow Bus  LConnTagsString=a  ID=bus558  Vbase=500000  Vref=1  Vangle=0  VLF=1  angleLF=0
      settings: AttributesFormatString=|
      | %<ID>
      | %<Vbase>V
      | %<VLF>pu
      | %<angleLF>deg.
      | %<Name>
  bus559 : powerlib/Measurements/Load Flow Bus  LConnTagsString=a  ID=bus559  Vbase=500000  Vref=1  Vangle=0  VLF=1  angleLF=0
      settings: AttributesFormatString=|
      | %<ID>
      | %<Vbase>V
      | %<VLF>pu
      | %<angleLF>deg.
      | %<Name>
  bus56 : powerlib/Measurements/Load Flow Bus  LConnTagsString=a  ID=bus56  Vbase=138000  Vref=1  Vangle=0  VLF=1  angleLF=0
      settings: AttributesFormatString=|
      | %<ID>
      | %<Vbase>V
      | %<VLF>pu
      | %<angleLF>deg.
      | %<Name>
  bus560 : powerlib/Measurements/Load Flow Bus  LConnTagsString=a  ID=bus560  Vbase=500000  Vref=1  Vangle=0  VLF=1  angleLF=0
      settings: AttributesFormatString=|
      | %<ID>
      | %<Vbase>V
      | %<VLF>pu
      | %<angleLF>deg.
      | %<Name>
  bus561 : powerlib/Measurements/Load Flow Bus  LConnTagsString=a  ID=bus561  Vbase=500000  Vref=1  Vangle=0  VLF=1  angleLF=0
      settings: AttributesFormatString=|
      | %<ID>
      | %<Vbase>V
      | %<VLF>pu
      | %<angleLF>deg.
      | %<Name>
  bus562 : powerlib/Measurements/Load Flow Bus  LConnTagsString=a  ID=bus562  Vbase=500000  Vref=1  Vangle=0  VLF=1  angleLF=0
      settings: AttributesFormatString=|
      | %<ID>
      | %<Vbase>V
      | %<VLF>pu
      | %<angleLF>deg.
      | %<Name>
  bus563 : powerlib/Measurements/Load Flow Bus  LConnTagsString=a  ID=bus563  Vbase=500000  Vref=1  Vangle=0  VLF=1  angleLF=0
      settings: AttributesFormatString=|
      | %<ID>
      | %<Vbase>V
      | %<VLF>pu
      | %<angleLF>deg.
      | %<Name>
  bus564 : powerlib/Measurements/Load Flow Bus  LConnTagsString=a  ID=bus564  Vbase=500000  Vref=1  Vangle=0  VLF=1  angleLF=0
      settings: AttributesFormatString=|
      | %<ID>
      | %<Vbase>V
      | %<VLF>pu
      | %<angleLF>deg.
      | %<Name>
  bus565 : powerlib/Measurements/Load Flow Bus  LConnTagsString=a  ID=bus565  Vbase=500000  Vref=1  Vangle=0  VLF=1  angleLF=0
      settings: AttributesFormatString=|
      | %<ID>
      | %<Vbase>V
      | %<VLF>pu
      | %<angleLF>deg.
      | %<Name>
  bus566 : powerlib/Measurements/Load Flow Bus  LConnTagsString=a  ID=bus566  Vbase=500000  Vref=1  Vangle=0  VLF=1  angleLF=0
      settings: AttributesFormatString=|
      | %<ID>
      | %<Vbase>V
      | %<VLF>pu
      | %<angleLF>deg.
      | %<Name>
  bus567 : powerlib/Measurements/Load Flow Bus  LConnTagsString=a  ID=bus567  Vbase=500000  Vref=1  Vangle=0  VLF=1  angleLF=0
      settings: AttributesFormatString=|
      | %<ID>
      | %<Vbase>V
      | %<VLF>pu
      | %<angleLF>deg.
      | %<Name>
  bus568 : powerlib/Measurements/Load Flow Bus  LConnTagsString=a  ID=bus568  Vbase=500000  Vref=1  Vangle=0  VLF=1  angleLF=0
      settings: AttributesFormatString=|
      | %<ID>
      | %<Vbase>V
      | %<VLF>pu
      | %<angleLF>deg.
      | %<Name>
  bus569 : powerlib/Measurements/Load Flow Bus  LConnTagsString=a  ID=bus569  Vbase=500000  Vref=1  Vangle=0  VLF=1  angleLF=0
      settings: AttributesFormatString=|
      | %<ID>
      | %<Vbase>V
      | %<VLF>pu
      | %<angleLF>deg.
      | %<Name>
  bus57 : powerlib/Measurements/Load Flow Bus  LConnTagsString=a  ID=bus57  Vbase=138000  Vref=1  Vangle=0  VLF=1  angleLF=0
      settings: AttributesFormatString=|
      | %<ID>
      | %<Vbase>V
      | %<VLF>pu
      | %<angleLF>deg.
      | %<Name>
  bus570 : powerlib/Measurements/Load Flow Bus  LConnTagsString=a  ID=bus570  Vbase=500000  Vref=1  Vangle=0  VLF=1  angleLF=0
      settings: AttributesFormatString=|
      | %<ID>
      | %<Vbase>V
      | %<VLF>pu
      | %<angleLF>deg.
      | %<Name>
  bus571 : powerlib/Measurements/Load Flow Bus  LConnTagsString=a  ID=bus571  Vbase=500000  Vref=1  Vangle=0  VLF=1  angleLF=0
      settings: AttributesFormatString=|
      | %<ID>
      | %<Vbase>V
      | %<VLF>pu
      | %<angleLF>deg.
      | %<Name>
  bus572 : powerlib/Measurements/Load Flow Bus  LConnTagsString=a  ID=bus572  Vbase=500000  Vref=1  Vangle=0  VLF=1  angleLF=0
      settings: AttributesFormatString=|
      | %<ID>
      | %<Vbase>V
      | %<VLF>pu
      | %<angleLF>deg.
      | %<Name>
  bus573 : powerlib/Measurements/Load Flow Bus  LConnTagsString=a  ID=bus573  Vbase=500000  Vref=1  Vangle=0  VLF=1  angleLF=0
      settings: AttributesFormatString=|
      | %<ID>
      | %<Vbase>V
      | %<VLF>pu
      | %<angleLF>deg.
      | %<Name>
  bus574 : powerlib/Measurements/Load Flow Bus  LConnTagsString=a  ID=bus574  Vbase=500000  Vref=1  Vangle=0  VLF=1  angleLF=0
      settings: AttributesFormatString=|
      | %<ID>
      | %<Vbase>V
      | %<VLF>pu
      | %<angleLF>deg.
      | %<Name>
  bus575 : powerlib/Measurements/Load Flow Bus  LConnTagsString=a  ID=bus575  Vbase=500000  Vref=1  Vangle=0  VLF=1  angleLF=0
      settings: AttributesFormatString=|
      | %<ID>
      | %<Vbase>V
      | %<VLF>pu
      | %<angleLF>deg.
      | %<Name>
  bus576 : powerlib/Measurements/Load Flow Bus  LConnTagsString=a  ID=bus576  Vbase=500000  Vref=1  Vangle=0  VLF=1  angleLF=0
      settings: AttributesFormatString=|
      | %<ID>
      | %<Vbase>V
      | %<VLF>pu
      | %<angleLF>deg.
      | %<Name>
  bus577 : powerlib/Measurements/Load Flow Bus  LConnTagsString=a  ID=bus577  Vbase=500000  Vref=1  Vangle=0  VLF=1  angleLF=0
      settings: AttributesFormatString=|
      | %<ID>
      | %<Vbase>V
      | %<VLF>pu
      | %<angleLF>deg.
      | %<Name>
  bus578 : powerlib/Measurements/Load Flow Bus  LConnTagsString=a  ID=bus578  Vbase=500000  Vref=1  Vangle=0  VLF=1  angleLF=0
      settings: AttributesFormatString=|
      | %<ID>
      | %<Vbase>V
      | %<VLF>pu
      | %<angleLF>deg.
      | %<Name>
  bus579 : powerlib/Measurements/Load Flow Bus  LConnTagsString=a  ID=bus579  Vbase=750000  Vref=1  Vangle=0  VLF=1  angleLF=0
      settings: AttributesFormatString=|
      | %<ID>
      | %<Vbase>V
      | %<VLF>pu
      | %<angleLF>deg.
      | %<Name>
  bus58 : powerlib/Measurements/Load Flow Bus  LConnTagsString=a  ID=bus58  Vbase=138000  Vref=1  Vangle=0  VLF=1  angleLF=0
      settings: AttributesFormatString=|
      | %<ID>
      | %<Vbase>V
      | %<VLF>pu
      | %<angleLF>deg.
      | %<Name>
  bus59 : powerlib/Measurements/Load Flow Bus  LConnTagsString=a  ID=bus59  Vbase=138000  Vref=1  Vangle=0  VLF=1  angleLF=0
      settings: AttributesFormatString=|
      | %<ID>
      | %<Vbase>V
      | %<VLF>pu
      | %<angleLF>deg.
      | %<Name>
  bus6 : powerlib/Measurements/Load Flow Bus  LConnTagsString=a  ID=bus6  Vbase=138000  Vref=1  Vangle=0  VLF=1  angleLF=0
      settings: AttributesFormatString=|
      | %<ID>
      | %<Vbase>V
      | %<VLF>pu
      | %<angleLF>deg.
      | %<Name>
  bus60 : powerlib/Measurements/Load Flow Bus  LConnTagsString=a  ID=bus60  Vbase=138000  Vref=1  Vangle=0  VLF=1  angleLF=0
      settings: AttributesFormatString=|
      | %<ID>
      | %<Vbase>V
      | %<VLF>pu
      | %<angleLF>deg.
      | %<Name>
  bus61 : powerlib/Measurements/Load Flow Bus  LConnTagsString=a  ID=bus61  Vbase=138000  Vref=1  Vangle=0  VLF=1  angleLF=0
      settings: AttributesFormatString=|
      | %<ID>
      | %<Vbase>V
      | %<VLF>pu
      | %<angleLF>deg.
      | %<Name>
  bus62 : powerlib/Measurements/Load Flow Bus  LConnTagsString=a  ID=bus62  Vbase=138000  Vref=1  Vangle=0  VLF=1  angleLF=0
      settings: AttributesFormatString=|
      | %<ID>
      | %<Vbase>V
      | %<VLF>pu
      | %<angleLF>deg.
      | %<Name>
  bus63 : powerlib/Measurements/Load Flow Bus  LConnTagsString=a  ID=bus63  Vbase=138000  Vref=1  Vangle=0  VLF=1  angleLF=0
      settings: AttributesFormatString=|
      | %<ID>
      | %<Vbase>V
      | %<VLF>pu
      | %<angleLF>deg.
      | %<Name>
  bus64 : powerlib/Measurements/Load Flow Bus  LConnTagsString=a  ID=bus64  Vbase=138000  Vref=1  Vangle=0  VLF=1  angleLF=0
      settings: AttributesFormatString=|
      | %<ID>
      | %<Vbase>V
      | %<VLF>pu
      | %<angleLF>deg.
      | %<Name>
  bus65 : powerlib/Measurements/Load Flow Bus  LConnTagsString=a  ID=bus65  Vbase=138000  Vref=1  Vangle=0  VLF=1  angleLF=0
      settings: AttributesFormatString=|
      | %<ID>
      | %<Vbase>V
      | %<VLF>pu
      | %<angleLF>deg.
      | %<Name>
  bus66 : powerlib/Measurements/Load Flow Bus  LConnTagsString=a  ID=bus66  Vbase=138000  Vref=1  Vangle=0  VLF=1  angleLF=0
      settings: AttributesFormatString=|
      | %<ID>
      | %<Vbase>V
      | %<VLF>pu
      | %<angleLF>deg.
      | %<Name>
  bus67 : powerlib/Measurements/Load Flow Bus  LConnTagsString=a  ID=bus67  Vbase=138000  Vref=1  Vangle=0  VLF=1  angleLF=0
      settings: AttributesFormatString=|
      | %<ID>
      | %<Vbase>V
      | %<VLF>pu
      | %<angleLF>deg.
      | %<Name>
  bus68 : powerlib/Measurements/Load Flow Bus  LConnTagsString=a  ID=bus68  Vbase=138000  Vref=1  Vangle=0  VLF=1  angleLF=0
      settings: AttributesFormatString=|
      | %<ID>
      | %<Vbase>V
      | %<VLF>pu
      | %<angleLF>deg.
      | %<Name>
  bus69 : powerlib/Measurements/Load Flow Bus  LConnTagsString=a  ID=bus69  Vbase=138000  Vref=1  Vangle=0  VLF=1  angleLF=0
      settings: AttributesFormatString=|
      | %<ID>
      | %<Vbase>V
      | %<VLF>pu
      | %<angleLF>deg.
      | %<Name>
  bus7 : powerlib/Measurements/Load Flow Bus  LConnTagsString=a  ID=bus7  Vbase=138000  Vref=1  Vangle=0  VLF=1  angleLF=0
      settings: AttributesFormatString=|
      | %<ID>
      | %<Vbase>V
      | %<VLF>pu
      | %<angleLF>deg.
      | %<Name>
  bus70 : powerlib/Measurements/Load Flow Bus  LConnTagsString=a  ID=bus70  Vbase=138000  Vref=1  Vangle=0  VLF=1  angleLF=0
      settings: AttributesFormatString=|
      | %<ID>
      | %<Vbase>V
      | %<VLF>pu
      | %<angleLF>deg.
      | %<Name>
  bus71 : powerlib/Measurements/Load Flow Bus  LConnTagsString=a  ID=bus71  Vbase=138000  Vref=1  Vangle=0  VLF=1  angleLF=0
      settings: AttributesFormatString=|
      | %<ID>
      | %<Vbase>V
      | %<VLF>pu
      | %<angleLF>deg.
      | %<Name>
  bus72 : powerlib/Measurements/Load Flow Bus  LConnTagsString=a  ID=bus72  Vbase=138000  Vref=1  Vangle=0  VLF=1  angleLF=0
      settings: AttributesFormatString=|
      | %<ID>
      | %<Vbase>V
      | %<VLF>pu
      | %<angleLF>deg.
      | %<Name>
  bus73 : powerlib/Measurements/Load Flow Bus  LConnTagsString=a  ID=bus73  Vbase=138000  Vref=1  Vangle=0  VLF=1  angleLF=0
      settings: AttributesFormatString=|
      | %<ID>
      | %<Vbase>V
      | %<VLF>pu
      | %<angleLF>deg.
      | %<Name>
  bus74 : powerlib/Measurements/Load Flow Bus  LConnTagsString=a  ID=bus74  Vbase=138000  Vref=1  Vangle=0  VLF=1  angleLF=0
      settings: AttributesFormatString=|
      | %<ID>
      | %<Vbase>V
      | %<VLF>pu
      | %<angleLF>deg.
      | %<Name>
  bus75 : powerlib/Measurements/Load Flow Bus  LConnTagsString=a  ID=bus75  Vbase=138000  Vref=1  Vangle=0  VLF=1  angleLF=0
      settings: AttributesFormatString=|
      | %<ID>
      | %<Vbase>V
      | %<VLF>pu
      | %<angleLF>deg.
      | %<Name>
  bus76 : powerlib/Measurements/Load Flow Bus  LConnTagsString=a  ID=bus76  Vbase=138000  Vref=1  Vangle=0  VLF=1  angleLF=0
      settings: AttributesFormatString=|
      | %<ID>
      | %<Vbase>V
      | %<VLF>pu
      | %<angleLF>deg.
      | %<Name>
  bus77 : powerlib/Measurements/Load Flow Bus  LConnTagsString=a  ID=bus77  Vbase=138000  Vref=1  Vangle=0  VLF=1  angleLF=0
      settings: AttributesFormatString=|
      | %<ID>
      | %<Vbase>V
      | %<VLF>pu
      | %<angleLF>deg.
      | %<Name>
  bus78 : powerlib/Measurements/Load Flow Bus  LConnTagsString=a  ID=bus78  Vbase=138000  Vref=1  Vangle=0  VLF=1  angleLF=0
      settings: AttributesFormatString=|
      | %<ID>
      | %<Vbase>V
      | %<VLF>pu
      | %<angleLF>deg.
      | %<Name>
  bus79 : powerlib/Measurements/Load Flow Bus  LConnTagsString=a  ID=bus79  Vbase=138000  Vref=1  Vangle=0  VLF=1  angleLF=0
      settings: AttributesFormatString=|
      | %<ID>
      | %<Vbase>V
      | %<VLF>pu
      | %<angleLF>deg.
      | %<Name>
  bus8 : powerlib/Measurements/Load Flow Bus  LConnTagsString=a  ID=bus8  Vbase=138000  Vref=1  Vangle=0  VLF=1  angleLF=0
      settings: AttributesFormatString=|
      | %<ID>
      | %<Vbase>V
      | %<VLF>pu
      | %<angleLF>deg.
      | %<Name>
  bus80 : powerlib/Measurements/Load Flow Bus  LConnTagsString=a  ID=bus80  Vbase=138000  Vref=1  Vangle=0  VLF=1  angleLF=0
      settings: AttributesFormatString=|
      | %<ID>
      | %<Vbase>V
      | %<VLF>pu
      | %<angleLF>deg.
      | %<Name>
  bus81 : powerlib/Measurements/Load Flow Bus  LConnTagsString=a  ID=bus81  Vbase=138000  Vref=1  Vangle=0  VLF=1  angleLF=0
      settings: AttributesFormatString=|
      | %<ID>
      | %<Vbase>V
      | %<VLF>pu
      | %<angleLF>deg.
      | %<Name>
  bus82 : powerlib/Measurements/Load Flow Bus  LConnTagsString=a  ID=bus82  Vbase=138000  Vref=1  Vangle=0  VLF=1  angleLF=0
      settings: AttributesFormatString=|
      | %<ID>
      | %<Vbase>V
      | %<VLF>pu
      | %<angleLF>deg.
      | %<Name>
  bus83 : powerlib/Measurements/Load Flow Bus  LConnTagsString=a  ID=bus83  Vbase=138000  Vref=1  Vangle=0  VLF=1  angleLF=0
      settings: AttributesFormatString=|
      | %<ID>
      | %<Vbase>V
      | %<VLF>pu
      | %<angleLF>deg.
      | %<Name>
  bus84 : powerlib/Measurements/Load Flow Bus  LConnTagsString=a  ID=bus84  Vbase=138000  Vref=1  Vangle=0  VLF=1  angleLF=0
      settings: AttributesFormatString=|
      | %<ID>
      | %<Vbase>V
      | %<VLF>pu
      | %<angleLF>deg.
      | %<Name>
  bus85 : powerlib/Measurements/Load Flow Bus  LConnTagsString=a  ID=bus85  Vbase=230000  Vref=1  Vangle=0  VLF=1  angleLF=0
      settings: AttributesFormatString=|
      | %<ID>
      | %<Vbase>V
      | %<VLF>pu
      | %<angleLF>deg.
      | %<Name>
  bus86 : powerlib/Measurements/Load Flow Bus  LConnTagsString=a  ID=bus86  Vbase=230000  Vref=1  Vangle=0  VLF=1  angleLF=0
      settings: AttributesFormatString=|
      | %<ID>
      | %<Vbase>V
      | %<VLF>pu
      | %<angleLF>deg.
      | %<Name>
  bus87 : powerlib/Measurements/Load Flow Bus  LConnTagsString=a  ID=bus87  Vbase=230000  Vref=1  Vangle=0  VLF=1  angleLF=0
      settings: AttributesFormatString=|
      | %<ID>
      | %<Vbase>V
      | %<VLF>pu
      | %<angleLF>deg.
      | %<Name>
  bus88 : powerlib/Measurements/Load Flow Bus  LConnTagsString=a  ID=bus88  Vbase=230000  Vref=1  Vangle=0  VLF=1  angleLF=0
      settings: AttributesFormatString=|
      | %<ID>
      | %<Vbase>V
      | %<VLF>pu
      | %<angleLF>deg.
      | %<Name>
  bus89 : powerlib/Measurements/Load Flow Bus  LConnTagsString=a  ID=bus89  Vbase=230000  Vref=1  Vangle=0  VLF=1  angleLF=0
      settings: AttributesFormatString=|
      | %<ID>
      | %<Vbase>V
      | %<VLF>pu
      | %<angleLF>deg.
      | %<Name>
  bus9 : powerlib/Measurements/Load Flow Bus  LConnTagsString=a  ID=bus9  Vbase=138000  Vref=1  Vangle=0  VLF=1  angleLF=0
      settings: AttributesFormatString=|
      | %<ID>
      | %<Vbase>V
      | %<VLF>pu
      | %<angleLF>deg.
      | %<Name>
  bus90 : powerlib/Measurements/Load Flow Bus  LConnTagsString=a  ID=bus90  Vbase=230000  Vref=1  Vangle=0  VLF=1  angleLF=0
      settings: AttributesFormatString=|
      | %<ID>
      | %<Vbase>V
      | %<VLF>pu
      | %<angleLF>deg.
      | %<Name>
  bus91 : powerlib/Measurements/Load Flow Bus  LConnTagsString=a  ID=bus91  Vbase=230000  Vref=1  Vangle=0  VLF=1  angleLF=0
      settings: AttributesFormatString=|
      | %<ID>
      | %<Vbase>V
      | %<VLF>pu
      | %<angleLF>deg.
      | %<Name>
  bus92 : powerlib/Measurements/Load Flow Bus  LConnTagsString=a  ID=bus92  Vbase=230000  Vref=1  Vangle=0  VLF=1  angleLF=0
      settings: AttributesFormatString=|
      | %<ID>
      | %<Vbase>V
      | %<VLF>pu
      | %<angleLF>deg.
      | %<Name>
  bus93 : powerlib/Measurements/Load Flow Bus  LConnTagsString=a  ID=bus93  Vbase=230000  Vref=1  Vangle=0  VLF=1  angleLF=0
      settings: AttributesFormatString=|
      | %<ID>
      | %<Vbase>V
      | %<VLF>pu
      | %<angleLF>deg.
      | %<Name>
  bus94 : powerlib/Measurements/Load Flow Bus  LConnTagsString=a  ID=bus94  Vbase=230000  Vref=1  Vangle=0  VLF=1  angleLF=0
      settings: AttributesFormatString=|
      | %<ID>
      | %<Vbase>V
      | %<VLF>pu
      | %<angleLF>deg.
      | %<Name>
  bus95 : powerlib/Measurements/Load Flow Bus  LConnTagsString=a  ID=bus95  Vbase=230000  Vref=1  Vangle=0  VLF=1  angleLF=0
      settings: AttributesFormatString=|
      | %<ID>
      | %<Vbase>V
      | %<VLF>pu
      | %<angleLF>deg.
      | %<Name>
  bus96 : powerlib/Measurements/Load Flow Bus  LConnTagsString=a  ID=bus96  Vbase=230000  Vref=1  Vangle=0  VLF=1  angleLF=0
      settings: AttributesFormatString=|
      | %<ID>
      | %<Vbase>V
      | %<VLF>pu
      | %<angleLF>deg.
      | %<Name>
  bus97 : powerlib/Measurements/Load Flow Bus  LConnTagsString=a  ID=bus97  Vbase=230000  Vref=1  Vangle=0  VLF=1  angleLF=0
      settings: AttributesFormatString=|
      | %<ID>
      | %<Vbase>V
      | %<VLF>pu
      | %<angleLF>deg.
      | %<Name>
  bus98 : powerlib/Measurements/Load Flow Bus  LConnTagsString=a  ID=bus98  Vbase=230000  Vref=1  Vangle=0  VLF=1  angleLF=0
      settings: AttributesFormatString=|
      | %<ID>
      | %<Vbase>V
      | %<VLF>pu
      | %<angleLF>deg.
      | %<Name>
  bus99 : powerlib/Measurements/Load Flow Bus  LConnTagsString=a  ID=bus99  Vbase=230000  Vref=1  Vangle=0  VLF=1  angleLF=0
      settings: AttributesFormatString=|
      | %<ID>
      | %<Vbase>V
      | %<VLF>pu
      | %<angleLF>deg.
      | %<Name>
  powergui : powerlib/powergui  Priority=1  SimulationMode=Continuous  SolverType=Tustin  SampleTime=50e-6  frequency=60  SPID=off  DisableSnubberDevices=off  DisableRonSwitches=off  DisableVfSwitches=off  SwTol=0  Interpol=off  DisplayEquations=off  Ts=0  methode=off  frequencyindice=60  Pbase=100e6  ErrMax=1e-4  Iterations=50  UnitsV=kV  UnitsW=MW  FunctionMessages=off  echomessages=off  HookPort=off  EnableUseOfTLC=off  x0status=blocks  RestoreLinks=warning  ResistiveCurrentMeasurement=off  Frange=[0:2:500]  Ylog=off  Xlog=on  ShowGrid=off  save=off  variable=ZData  structure=0  ZoomFFT=off  StartTime=0.0  cycles=1  DisplayStyle=1  fundamental=60  FreqAxis=off  MaxFrequency=1000  frequencyindicesteady=1  RmsSteady=1  display=off
  connections:
  T_204662228__/LConn1 -- _CN_204662228_138000_CN_208450687_138000/LConn1
  T_204662228__/LConn2 -- _CN_204662228_138000_CN_208450687_138000/LConn2
  _CN_204662228_138000_CN_208450687_138000/LConn3 -- T_204662228__/LConn3 -- bus1/LConn1
  _CN_204662228_138000_CN_208450687_138000/RConn1 -- T_208450687__Subestação_COPEL_Toledo/LConn1 -- Linha_de_Transmissão_Toledo_Marechal_CN_207573521_138000_CN_208450687_138000/LConn1
  _CN_204662228_138000_CN_208450687_138000/RConn2 -- T_208450687__Subestação_COPEL_Toledo/LConn2 -- Linha_de_Transmissão_Toledo_Marechal_CN_207573521_138000_CN_208450687_138000/LConn2
  _CN_204662228_138000_CN_208450687_138000/RConn3 -- T_208450687__Subestação_COPEL_Toledo/LConn3 -- Linha_de_Transmissão_Toledo_Marechal_CN_207573521_138000_CN_208450687_138000/LConn3 -- bus2/LConn1
  T_207573521__/LConn1 -- Linha_de_Transmissão_Toledo_Marechal_CN_207573521_138000_CN_208450687_138000/RConn1
  T_207573521__/LConn2 -- Linha_de_Transmissão_Toledo_Marechal_CN_207573521_138000_CN_208450687_138000/RConn2
  Linha_de_Transmissão_Toledo_Marechal_CN_207573521_138000_CN_208450687_138000/RConn3 -- T_207573521__/LConn3 -- bus3/LConn1
  T_430397465__Subestação_Rio_Azul/LConn1 -- Linha_SE_Irati_SE_Rio_Azul_CN_430397465_138000_CN_430390206_138000/LConn1
  T_430397465__Subestação_Rio_Azul/LConn2 -- Linha_SE_Irati_SE_Rio_Azul_CN_430397465_138000_CN_430390206_138000/LConn2
  Linha_SE_Irati_SE_Rio_Azul_CN_430397465_138000_CN_430390206_138000/LConn3 -- T_430397465__Subestação_Rio_Azul/LConn3 -- bus4/LConn1
  Linha_SE_Irati_SE_Rio_Azul_CN_430397465_138000_CN_430390206_138000/RConn1 -- T_430390206__Subestação_Irati/LConn1 -- Linha_SE_Guarapuava_SE_Irati_CN_430385951_138000_CN_430390206_138000/LConn1 -- Linha_SE_Irati_SE_Sabará_CN_430403964_138000_CN_430390206_138000/LConn1
  Linha_SE_Irati_SE_Rio_Azul_CN_430397465_138000_CN_430390206_138000/RConn2 -- T_430390206__Subestação_Irati/LConn2 -- Linha_SE_Guarapuava_SE_Irati_CN_430385951_138000_CN_430390206_138000/LConn2 -- Linha_SE_Irati_SE_Sabará_CN_430403964_138000_CN_430390206_138000/LConn2
  Linha_SE_Irati_SE_Rio_Azul_CN_430397465_138000_CN_430390206_138000/RConn3 -- T_430390206__Subestação_Irati/LConn3 -- Linha_SE_Guarapuava_SE_Irati_CN_430385951_138000_CN_430390206_138000/LConn3 -- Linha_SE_Irati_SE_Sabará_CN_430403964_138000_CN_430390206_138000/LConn3 -- bus5/LConn1
  T_171490852__Subestação_Parque_das_Emas/LConn1 -- _CN_171490852_138000_CN_174643089_138000/LConn1
  T_171490852__Subestação_Parque_das_Emas/LConn2 -- _CN_171490852_138000_CN_174643089_138000/LConn2
  _CN_171490852_138000_CN_174643089_138000/LConn3 -- T_171490852__Subestação_Parque_das_Emas/LConn3 -- bus6/LConn1
  _CN_171490852_138000_CN_174643089_138000/RConn1 -- T_174643089__Rio_Verde/RConn1 -- L_174643089/LConn1
  _CN_171490852_138000_CN_174643089_138000/RConn2 -- T_174643089__Rio_Verde/RConn2 -- L_174643089/LConn2
  _CN_171490852_138000_CN_174643089_138000/RConn3 -- T_174643089__Rio_Verde/RConn3 -- L_174643089/LConn3 -- bus7/LConn1
  T_238221864__Subestação_Chapecó_II/LConn1 -- _CN_238221864_138000_CN_206686475_138000/LConn1
  T_238221864__Subestação_Chapecó_II/LConn2 -- _CN_238221864_138000_CN_206686475_138000/LConn2
  _CN_238221864_138000_CN_206686475_138000/LConn3 -- T_238221864__Subestação_Chapecó_II/LConn3 -- bus8/LConn1
  T_206686475_138000_Subestação_Xanxerê_Celesc/LConn1 -- _CN_238221864_138000_CN_206686475_138000/RConn1
  T_206686475_138000_Subestação_Xanxerê_Celesc/LConn2 -- _CN_238221864_138000_CN_206686475_138000/RConn2
  _CN_238221864_138000_CN_206686475_138000/RConn3 -- T_206686475_138000_Subestação_Xanxerê_Celesc/LConn3 -- bus9/LConn1
  T_206721069__Subestação_BRF/LConn1 -- Linha_de_Transmissão_Frigobrás_Toledo_Cascavel_CN_206721069_138000_CN_361161020_138000/LConn1
  T_206721069__Subestação_BRF/LConn2 -- Linha_de_Transmissão_Frigobrás_Toledo_Cascavel_CN_206721069_138000_CN_361161020_138000/LConn2
  Linha_de_Transmissão_Frigobrás_Toledo_Cascavel_CN_206721069_138000_CN_361161020_138000/LConn3 -- T_206721069__Subestação_BRF/LConn3 -- bus10/LConn1
  T_361161020__/LConn1 -- Linha_de_Transmissão_Frigobrás_Toledo_Cascavel_CN_206721069_138000_CN_361161020_138000/RConn1
  T_361161020__/LConn2 -- Linha_de_Transmissão_Frigobrás_Toledo_Cascavel_CN_206721069_138000_CN_361161020_138000/RConn2
  Linha_de_Transmissão_Frigobrás_Toledo_Cascavel_CN_206721069_138000_CN_361161020_138000/RConn3 -- T_361161020__/LConn3 -- bus11/LConn1
  _CN_166830130_138000_CN_108479345_138000/LConn1 -- T_166830130__/LConn1 -- _CN_166830130_138000_CN_283714330_138000/LConn1
  _CN_166830130_138000_CN_108479345_138000/LConn2 -- T_166830130__/LConn2 -- _CN_166830130_138000_CN_283714330_138000/LConn2
  _CN_166830130_138000_CN_108479345_138000/LConn3 -- T_166830130__/LConn3 -- _CN_166830130_138000_CN_283714330_138000/LConn3 -- bus12/LConn1
  T_108479345__/LConn1 -- _CN_166830130_138000_CN_108479345_138000/RConn1
  T_108479345__/LConn2 -- _CN_166830130_138000_CN_108479345_138000/RConn2
  _CN_166830130_138000_CN_108479345_138000/RConn3 -- T_108479345__/LConn3 -- bus13/LConn1
  T_283714330__/LConn1 -- _CN_166830130_138000_CN_283714330_138000/RConn1
  T_283714330__/LConn2 -- _CN_166830130_138000_CN_283714330_138000/RConn2
  _CN_166830130_138000_CN_283714330_138000/RConn3 -- T_283714330__/LConn3 -- bus14/LConn1
  T_109816378__/LConn1 -- _CN_109816378_138000_CN_421202632_138000/LConn1
  T_109816378__/LConn2 -- _CN_109816378_138000_CN_421202632_138000/LConn2
  _CN_109816378_138000_CN_421202632_138000/LConn3 -- T_109816378__/LConn3 -- bus15/LConn1
  _CN_109816378_138000_CN_421202632_138000/RConn1 -- T_421202632__Subestação_Jorge_Lacerda_B/RConn1 -- L_421202632/LConn1
  _CN_109816378_138000_CN_421202632_138000/RConn2 -- T_421202632__Subestação_Jorge_Lacerda_B/RConn2 -- L_421202632/LConn2
  _CN_109816378_138000_CN_421202632_138000/RConn3 -- T_421202632__Subestação_Jorge_Lacerda_B/RConn3 -- L_421202632/LConn3 -- bus16/LConn1
  T_179031106__/LConn1 -- _CN_179031106_138000_CN_180585890_138000/LConn1
  T_179031106__/LConn2 -- _CN_179031106_138000_CN_180585890_138000/LConn2
  _CN_179031106_138000_CN_180585890_138000/LConn3 -- T_179031106__/LConn3 -- bus17/LConn1
  T_180585890_138000_/LConn1 -- _CN_179031106_138000_CN_180585890_138000/RConn1
  T_180585890_138000_/LConn2 -- _CN_179031106_138000_CN_180585890_138000/RConn2
  _CN_179031106_138000_CN_180585890_138000/RConn3 -- T_180585890_138000_/LConn3 -- bus18/LConn1
  T_258563660__/LConn1 -- _CN_258563660_138000_CN_168692156_138000/LConn1
  T_258563660__/LConn2 -- _CN_258563660_138000_CN_168692156_138000/LConn2
  _CN_258563660_138000_CN_168692156_138000/LConn3 -- T_258563660__/LConn3 -- bus19/LConn1
  _CN_258563660_138000_CN_168692156_138000/RConn1 -- T_168692156__Furnas/RConn1 -- _CN_154646743_138000_CN_168692156_138000/LConn1 -- _CN_168692156_138000_CN_168692185_138000/LConn1 -- L_168692156/LConn1
  _CN_258563660_138000_CN_168692156_138000/RConn2 -- T_168692156__Furnas/RConn2 -- _CN_154646743_138000_CN_168692156_138000/LConn2 -- _CN_168692156_138000_CN_168692185_138000/LConn2 -- L_168692156/LConn2
  _CN_258563660_138000_CN_168692156_138000/RConn3 -- T_168692156__Furnas/RConn3 -- _CN_154646743_138000_CN_168692156_138000/LConn3 -- _CN_168692156_138000_CN_168692185_138000/LConn3 -- L_168692156/LConn3 -- bus20/LConn1
  T_374370399__/LConn1 -- _CN_374370399_138000_CN_215501231_138000/LConn1
  T_374370399__/LConn2 -- _CN_374370399_138000_CN_215501231_138000/LConn2
  _CN_374370399_138000_CN_215501231_138000/LConn3 -- T_374370399__/LConn3 -- bus21/LConn1
  _CN_374370399_138000_CN_215501231_138000/RConn1 -- T_215501231__/LConn1 -- _CN_173329706_138000_CN_215501231_138000/LConn1
  _CN_374370399_138000_CN_215501231_138000/RConn2 -- T_215501231__/LConn2 -- _CN_173329706_138000_CN_215501231_138000/LConn2
  _CN_374370399_138000_CN_215501231_138000/RConn3 -- T_215501231__/LConn3 -- _CN_173329706_138000_CN_215501231_138000/LConn3 -- bus22/LConn1
  T_169845345__Subestação_Rodoviária/LConn1 -- LT_CPA___Rodoviária___Cidade_Alta_CN_169845345_138000_CN_167892676_138000/LConn1
  T_169845345__Subestação_Rodoviária/LConn2 -- LT_CPA___Rodoviária___Cidade_Alta_CN_169845345_138000_CN_167892676_138000/LConn2
  LT_CPA___Rodoviária___Cidade_Alta_CN_169845345_138000_CN_167892676_138000/LConn3 -- T_169845345__Subestação_Rodoviária/LConn3 -- bus23/LConn1
  LT_CPA___Rodoviária___Cidade_Alta_CN_169845345_138000_CN_167892676_138000/RConn1 -- T_167892676__Subestação_CPA/LConn1 -- LT_UTE_Cuiabá___Coxipó_CN_167892676_138000_CN_320803018_138000/LConn1 -- LT_UTE_Cuiabá___Coxipó_CN_167892676_138000_CN_167284528_138000/LConn1
  LT_CPA___Rodoviária___Cidade_Alta_CN_169845345_138000_CN_167892676_138000/RConn2 -- T_167892676__Subestação_CPA/LConn2 -- LT_UTE_Cuiabá___Coxipó_CN_167892676_138000_CN_320803018_138000/LConn2 -- LT_UTE_Cuiabá___Coxipó_CN_167892676_138000_CN_167284528_138000/LConn2
  LT_CPA___Rodoviária___Cidade_Alta_CN_169845345_138000_CN_167892676_138000/RConn3 -- T_167892676__Subestação_CPA/LConn3 -- LT_UTE_Cuiabá___Coxipó_CN_167892676_138000_CN_320803018_138000/LConn3 -- bus24/LConn1 -- LT_UTE_Cuiabá___Coxipó_CN_167892676_138000_CN_167284528_138000/LConn3
  _CN_315151458_138000_CN_306133422_138000/LConn1 -- T_315151458__Daia/LConn1 -- _CN_315151458_138000_CN_291611826_138000/LConn1 -- _CN_315151458_138000_CN_315172147_138000/LConn1
  _CN_315151458_138000_CN_306133422_138000/LConn2 -- T_315151458__Daia/LConn2 -- _CN_315151458_138000_CN_291611826_138000/LConn2 -- _CN_315151458_138000_CN_315172147_138000/LConn2
  _CN_315151458_138000_CN_306133422_138000/LConn3 -- T_315151458__Daia/LConn3 -- _CN_315151458_138000_CN_291611826_138000/LConn3 -- _CN_315151458_138000_CN_315172147_138000/LConn3 -- bus25/LConn1
  _CN_315151458_138000_CN_306133422_138000/RConn1 -- T_306133422__Subestação_Anhanguera/RConn4 -- L_306133422/LConn1
  _CN_315151458_138000_CN_306133422_138000/RConn2 -- T_306133422__Subestação_Anhanguera/RConn5 -- L_306133422/LConn2
  _CN_315151458_138000_CN_306133422_138000/RConn3 -- T_306133422__Subestação_Anhanguera/RConn6 -- L_306133422/LConn3 -- bus26/LConn1
  _CN_315151458_138000_CN_291611826_138000/RConn1 -- T_291611826__Subestação_da_CELG/RConn1 -- _CN_313920196_138000_CN_291611826_138000/LConn1 -- L_291611826/LConn1
  _CN_315151458_138000_CN_291611826_138000/RConn2 -- T_291611826__Subestação_da_CELG/RConn2 -- _CN_313920196_138000_CN_291611826_138000/LConn2 -- L_291611826/LConn2
  _CN_315151458_138000_CN_291611826_138000/RConn3 -- T_291611826__Subestação_da_CELG/RConn3 -- _CN_313920196_138000_CN_291611826_138000/LConn3 -- L_291611826/LConn3 -- bus27/LConn1
  T_315172147__/LConn1 -- _CN_315151458_138000_CN_315172147_138000/RConn1
  T_315172147__/LConn2 -- _CN_315151458_138000_CN_315172147_138000/RConn2
  _CN_315151458_138000_CN_315172147_138000/RConn3 -- T_315172147__/LConn3 -- bus28/LConn1
  T_168904821__Jauru/LConn1 -- _CN_168904821_138000_CN_168904844_138000/LConn1
  T_168904821__Jauru/LConn2 -- _CN_168904821_138000_CN_168904844_138000/LConn2
  _CN_168904821_138000_CN_168904844_138000/LConn3 -- T_168904821__Jauru/LConn3 -- bus29/LConn1
  _CN_168904821_138000_CN_168904844_138000/RConn1 -- T_168904844__Subestação_Jauru/RConn1 -- _CN_168904839_138000_CN_168904844_138000/LConn1 -- _CN_168904844_138000_CN_168933874_138000/LConn1 -- L_168904844/LConn1
  _CN_168904821_138000_CN_168904844_138000/RConn2 -- T_168904844__Subestação_Jauru/RConn2 -- _CN_168904839_138000_CN_168904844_138000/LConn2 -- _CN_168904844_138000_CN_168933874_138000/LConn2 -- L_168904844/LConn2
  _CN_168904821_138000_CN_168904844_138000/RConn3 -- T_168904844__Subestação_Jauru/RConn3 -- _CN_168904839_138000_CN_168904844_138000/LConn3 -- _CN_168904844_138000_CN_168933874_138000/LConn3 -- L_168904844/LConn3 -- bus30/LConn1
  T_306676350__Subestação_Batávia/LConn1 -- Linha_Ponta_Grossa_Norte___Batávia_CN_306676350_138000_CN_306588466_138000/LConn1
  T_306676350__Subestação_Batávia/LConn2 -- Linha_Ponta_Grossa_Norte___Batávia_CN_306676350_138000_CN_306588466_138000/LConn2
  Linha_Ponta_Grossa_Norte___Batávia_CN_306676350_138000_CN_306588466_138000/LConn3 -- T_306676350__Subestação_Batávia/LConn3 -- bus31/LConn1
  Linha_Ponta_Grossa_Norte___Batávia_CN_306676350_138000_CN_306588466_138000/RConn1 -- T_306588466__Subestação_Ponta_Grossa_Norte/RConn1 -- Linha_SE_Ponta_Grossa_Norte_SE_Sabará_CN_306588466_138000_CN_430403964_138000/LConn1 -- L_306588466/LConn1
  Linha_Ponta_Grossa_Norte___Batávia_CN_306676350_138000_CN_306588466_138000/RConn2 -- T_306588466__Subestação_Ponta_Grossa_Norte/RConn2 -- Linha_SE_Ponta_Grossa_Norte_SE_Sabará_CN_306588466_138000_CN_430403964_138000/LConn2 -- L_306588466/LConn2
  Linha_Ponta_Grossa_Norte___Batávia_CN_306676350_138000_CN_306588466_138000/RConn3 -- T_306588466__Subestação_Ponta_Grossa_Norte/RConn3 -- Linha_SE_Ponta_Grossa_Norte_SE_Sabará_CN_306588466_138000_CN_430403964_138000/LConn3 -- L_306588466/LConn3 -- bus32/LConn1
  T_168904839__Subestação_Guaporé/LConn1 -- _CN_168904839_138000_CN_168904844_138000/RConn1
  T_168904839__Subestação_Guaporé/LConn2 -- _CN_168904839_138000_CN_168904844_138000/RConn2
  _CN_168904839_138000_CN_168904844_138000/RConn3 -- T_168904839__Subestação_Guaporé/LConn3 -- bus33/LConn1
  T_168933874__/LConn1 -- _CN_168904844_138000_CN_168933874_138000/RConn1
  T_168933874__/LConn2 -- _CN_168904844_138000_CN_168933874_138000/RConn2
  _CN_168904844_138000_CN_168933874_138000/RConn3 -- T_168933874__/LConn3 -- bus34/LConn1
  _CN_41756817_138000_CN_290054123_138000/LConn1 -- T_41756817__Cidade_Industrial/RConn1 -- L_41756817/LConn1
  _CN_41756817_138000_CN_290054123_138000/LConn2 -- T_41756817__Cidade_Industrial/RConn2 -- L_41756817/LConn2
  _CN_41756817_138000_CN_290054123_138000/LConn3 -- T_41756817__Cidade_Industrial/RConn3 -- L_41756817/LConn3 -- bus35/LConn1
  T_290054123__São_Luís/LConn1 -- _CN_41756817_138000_CN_290054123_138000/RConn1
  T_290054123__São_Luís/LConn2 -- _CN_41756817_138000_CN_290054123_138000/RConn2
  _CN_41756817_138000_CN_290054123_138000/RConn3 -- T_290054123__São_Luís/LConn3 -- bus36/LConn1
  _CN_288144022_138000_CN_315069128_138000/LConn1 -- T_288144022__/LConn1 -- _CN_288144022_138000_CN_286116282_138000/LConn1
  _CN_288144022_138000_CN_315069128_138000/LConn2 -- T_288144022__/LConn2 -- _CN_288144022_138000_CN_286116282_138000/LConn2
  _CN_288144022_138000_CN_315069128_138000/LConn3 -- T_288144022__/LConn3 -- _CN_288144022_138000_CN_286116282_138000/LConn3 -- bus37/LConn1
  T_315069128__Jundiai/LConn1 -- _CN_288144022_138000_CN_315069128_138000/RConn1
  T_315069128__Jundiai/LConn2 -- _CN_288144022_138000_CN_315069128_138000/RConn2
  _CN_288144022_138000_CN_315069128_138000/RConn3 -- T_315069128__Jundiai/LConn3 -- bus38/LConn1
  T_286116282__/LConn1 -- _CN_288144022_138000_CN_286116282_138000/RConn1
  T_286116282__/LConn2 -- _CN_288144022_138000_CN_286116282_138000/RConn2
  _CN_288144022_138000_CN_286116282_138000/RConn3 -- T_286116282__/LConn3 -- bus39/LConn1
  T_313920196__/LConn1 -- _CN_313920196_138000_CN_291611826_138000/RConn1
  T_313920196__/LConn2 -- _CN_313920196_138000_CN_291611826_138000/RConn2
  _CN_313920196_138000_CN_291611826_138000/RConn3 -- T_313920196__/LConn3 -- bus40/LConn1
  _CN_108198075_138000_CN_108224468_138000/LConn1 -- T_108198075__Subestação_Jacarepaguá/RConn1 -- _CN_108198075_138000_CN_108435010_138000/LConn1 -- L_108198075/LConn1 -- _CN_108198075_138000_CN_116704519_138000/LConn1
  _CN_108198075_138000_CN_108224468_138000/LConn2 -- T_108198075__Subestação_Jacarepaguá/RConn2 -- _CN_108198075_138000_CN_108435010_138000/LConn2 -- L_108198075/LConn2 -- _CN_108198075_138000_CN_116704519_138000/LConn2
  _CN_108198075_138000_CN_108224468_138000/LConn3 -- T_108198075__Subestação_Jacarepaguá/RConn3 -- _CN_108198075_138000_CN_108435010_138000/LConn3 -- L_108198075/LConn3 -- bus41/LConn1 -- _CN_108198075_138000_CN_116704519_138000/LConn3
  _CN_108198075_138000_CN_108224468_138000/RConn1 -- T_108224468_500000_Subestação_Grajaú/RConn1 -- _CN_122252210_138000_CN_108224468_138000/LConn1 -- _CN_122252211_138000_CN_108224468_138000/LConn1 -- _CN_108435903_138000_CN_108224468_138000/LConn1 -- L_108224468/LConn1
  _CN_108198075_138000_CN_108224468_138000/RConn2 -- T_108224468_500000_Subestação_Grajaú/RConn2 -- _CN_122252210_138000_CN_108224468_138000/LConn2 -- _CN_122252211_138000_CN_108224468_138000/LConn2 -- _CN_108435903_138000_CN_108224468_138000/LConn2 -- L_108224468/LConn2
  _CN_108198075_138000_CN_108224468_138000/RConn3 -- T_108224468_500000_Subestação_Grajaú/RConn3 -- _CN_122252210_138000_CN_108224468_138000/LConn3 -- _CN_122252211_138000_CN_108224468_138000/LConn3 -- _CN_108435903_138000_CN_108224468_138000/LConn3 -- L_108224468/LConn3 -- bus42/LConn1
  G_116704519_/RConn1 -- _CN_108198075_138000_CN_116704519_138000/RConn1
  G_116704519_/RConn2 -- _CN_108198075_138000_CN_116704519_138000/RConn2
  _CN_108198075_138000_CN_116704519_138000/RConn3 -- G_116704519_/RConn3 -- bus43/LConn1
  T_108435010__/LConn1 -- _CN_108198075_138000_CN_108435010_138000/RConn1
  T_108435010__/LConn2 -- _CN_108198075_138000_CN_108435010_138000/RConn2
  _CN_108198075_138000_CN_108435010_138000/RConn3 -- T_108435010__/LConn3 -- bus44/LConn1
  T_179642046__Subestação_Mourão/LConn1 -- _CN_179642046_138000_CN_394083271_138000/LConn1
  T_179642046__Subestação_Mourão/LConn2 -- _CN_179642046_138000_CN_394083271_138000/LConn2
  _CN_179642046_138000_CN_394083271_138000/LConn3 -- T_179642046__Subestação_Mourão/LConn3 -- bus45/LConn1
  _CN_179642046_138000_CN_394083271_138000/RConn1 -- T_394083271_230000;13800_Subestação_Campo_Mourão/RConn1 -- _CN_395653952_138000_CN_394083271_138000/LConn1 -- _CN_395653957_138000_CN_394083271_138000/LConn1 -- L_394083271/LConn1
  _CN_179642046_138000_CN_394083271_138000/RConn2 -- T_394083271_230000;13800_Subestação_Campo_Mourão/RConn2 -- _CN_395653952_138000_CN_394083271_138000/LConn2 -- _CN_395653957_138000_CN_394083271_138000/LConn2 -- L_394083271/LConn2
  _CN_179642046_138000_CN_394083271_138000/RConn3 -- T_394083271_230000;13800_Subestação_Campo_Mourão/RConn3 -- _CN_395653952_138000_CN_394083271_138000/LConn3 -- _CN_395653957_138000_CN_394083271_138000/LConn3 -- L_394083271/LConn3 -- bus46/LConn1
  LT_UTE_Cuiabá___Coxipó_CN_167892676_138000_CN_167284528_138000/RConn1 -- T_167284528__Subestação_EPE/LConn1 -- LT_Várzea_Grande___EPE_CN_167284528_138000_CN_32957294_138000/LConn1
  LT_UTE_Cuiabá___Coxipó_CN_167892676_138000_CN_167284528_138000/RConn2 -- T_167284528__Subestação_EPE/LConn2 -- LT_Várzea_Grande___EPE_CN_167284528_138000_CN_32957294_138000/LConn2
  LT_UTE_Cuiabá___Coxipó_CN_167892676_138000_CN_167284528_138000/RConn3 -- T_167284528__Subestação_EPE/LConn3 -- LT_Várzea_Grande___EPE_CN_167284528_138000_CN_32957294_138000/LConn3 -- bus47/LConn1
  LT_UTE_Cuiabá___Coxipó_CN_167892676_138000_CN_320803018_138000/RConn1 -- T_320803018__Subestação_Coxipó/RConn1 -- LT_Rondonópolis___Coxipó_CN_320803018_138000_CN_45415932_138000/LConn1 -- L_320803018/LConn1
  LT_UTE_Cuiabá___Coxipó_CN_167892676_138000_CN_320803018_138000/RConn2 -- T_320803018__Subestação_Coxipó/RConn2 -- LT_Rondonópolis___Coxipó_CN_320803018_138000_CN_45415932_138000/LConn2 -- L_320803018/LConn2
  LT_UTE_Cuiabá___Coxipó_CN_167892676_138000_CN_320803018_138000/RConn3 -- T_320803018__Subestação_Coxipó/RConn3 -- LT_Rondonópolis___Coxipó_CN_320803018_138000_CN_45415932_138000/LConn3 -- L_320803018/LConn3 -- bus48/LConn1
  LT_Rondonópolis___Coxipó_CN_320803018_138000_CN_45415932_138000/RConn1 -- T_45415932__Subestação_Rondonópolis/RConn1 -- LT_Rio_Verde___Couto_Magalhães___Rondonópolis_CN_171490850_138000_CN_45415932_138000/LConn1 -- L_45415932/LConn1
  LT_Rondonópolis___Coxipó_CN_320803018_138000_CN_45415932_138000/RConn2 -- T_45415932__Subestação_Rondonópolis/RConn2 -- LT_Rio_Verde___Couto_Magalhães___Rondonópolis_CN_171490850_138000_CN_45415932_138000/LConn2 -- L_45415932/LConn2
  LT_Rondonópolis___Coxipó_CN_320803018_138000_CN_45415932_138000/RConn3 -- T_45415932__Subestação_Rondonópolis/RConn3 -- LT_Rio_Verde___Couto_Magalhães___Rondonópolis_CN_171490850_138000_CN_45415932_138000/LConn3 -- L_45415932/LConn3 -- bus49/LConn1
  T_171490850__Subestação_Couto_Magalhães/LConn1 -- LT_Rio_Verde___Couto_Magalhães___Rondonópolis_CN_171490850_138000_CN_45415932_138000/RConn1
  T_171490850__Subestação_Couto_Magalhães/LConn2 -- LT_Rio_Verde___Couto_Magalhães___Rondonópolis_CN_171490850_138000_CN_45415932_138000/RConn2
  LT_Rio_Verde___Couto_Magalhães___Rondonópolis_CN_171490850_138000_CN_45415932_138000/RConn3 -- T_171490850__Subestação_Couto_Magalhães/LConn3 -- bus50/LConn1
  T_199921358__/LConn1 -- _CN_199921358_138000_CN_199921360_138000/LConn1
  T_199921358__/LConn2 -- _CN_199921358_138000_CN_199921360_138000/LConn2
  _CN_199921358_138000_CN_199921360_138000/LConn3 -- T_199921358__/LConn3 -- bus51/LConn1
  _CN_199921358_138000_CN_199921360_138000/RConn1 -- T_199921360__/LConn1 -- _CN_199921360_138000_CN_200365032_138000/LConn1 -- _CN_199921360_138000_CN_194362821_138000/LConn1
  _CN_199921358_138000_CN_199921360_138000/RConn2 -- T_199921360__/LConn2 -- _CN_199921360_138000_CN_200365032_138000/LConn2 -- _CN_199921360_138000_CN_194362821_138000/LConn2
  _CN_199921358_138000_CN_199921360_138000/RConn3 -- T_199921360__/LConn3 -- _CN_199921360_138000_CN_200365032_138000/LConn3 -- _CN_199921360_138000_CN_194362821_138000/LConn3 -- bus52/LConn1
  T_200365032__/LConn1 -- _CN_199921360_138000_CN_200365032_138000/RConn1
  T_200365032__/LConn2 -- _CN_199921360_138000_CN_200365032_138000/RConn2
  _CN_199921360_138000_CN_200365032_138000/RConn3 -- T_200365032__/LConn3 -- bus53/LConn1
  T_194362821__Santa_Maria_1/LConn1 -- _CN_199921360_138000_CN_194362821_138000/RConn1
  T_194362821__Santa_Maria_1/LConn2 -- _CN_199921360_138000_CN_194362821_138000/RConn2
  _CN_199921360_138000_CN_194362821_138000/RConn3 -- T_194362821__Santa_Maria_1/LConn3 -- bus54/LConn1
  T_178582739__Subestação_Canarana/LConn1 -- LT_Canarana___Querência_CN_178582739_138000_CN_178582740_138000/LConn1
  T_178582739__Subestação_Canarana/LConn2 -- LT_Canarana___Querência_CN_178582739_138000_CN_178582740_138000/LConn2
  LT_Canarana___Querência_CN_178582739_138000_CN_178582740_138000/LConn3 -- T_178582739__Subestação_Canarana/LConn3 -- bus55/LConn1
  T_178582740__Subestação_Querência/LConn1 -- LT_Canarana___Querência_CN_178582739_138000_CN_178582740_138000/RConn1
  T_178582740__Subestação_Querência/LConn2 -- LT_Canarana___Querência_CN_178582739_138000_CN_178582740_138000/RConn2
  LT_Canarana___Querência_CN_178582739_138000_CN_178582740_138000/RConn3 -- T_178582740__Subestação_Querência/LConn3 -- bus56/LConn1
  T_154646743__/LConn1 -- _CN_154646743_138000_CN_168692156_138000/RConn1
  T_154646743__/LConn2 -- _CN_154646743_138000_CN_168692156_138000/RConn2
  _CN_154646743_138000_CN_168692156_138000/RConn3 -- T_154646743__/LConn3 -- bus57/LConn1
  _CN_256782575_138000_CN_256782585_138000/LConn1 -- T_256782575__Cachoeira_Dourada/RConn1 -- L_256782575/LConn1
  _CN_256782575_138000_CN_256782585_138000/LConn2 -- T_256782575__Cachoeira_Dourada/RConn2 -- L_256782575/LConn2
  _CN_256782575_138000_CN_256782585_138000/LConn3 -- T_256782575__Cachoeira_Dourada/RConn3 -- L_256782575/LConn3 -- bus58/LConn1
  T_256782585__/LConn1 -- _CN_256782575_138000_CN_256782585_138000/RConn1
  T_256782585__/LConn2 -- _CN_256782575_138000_CN_256782585_138000/RConn2
  _CN_256782575_138000_CN_256782585_138000/RConn3 -- T_256782585__/LConn3 -- bus59/LConn1
  T_176682224__Subestação_Cristo_Rei/LConn1 -- LT_Várzea_Grande___Cristo_Rei_CN_176682224_138000_CN_32957294_138000/LConn1
  T_176682224__Subestação_Cristo_Rei/LConn2 -- LT_Várzea_Grande___Cristo_Rei_CN_176682224_138000_CN_32957294_138000/LConn2
  LT_Várzea_Grande___Cristo_Rei_CN_176682224_138000_CN_32957294_138000/LConn3 -- T_176682224__Subestação_Cristo_Rei/LConn3 -- bus60/LConn1
  LT_Várzea_Grande___Cristo_Rei_CN_176682224_138000_CN_32957294_138000/RConn1 -- T_32957294__/LConn1 -- LT_Nobres___Várzea_Grande_CN_32957294_138000_CN_169406381_138000/LConn1 -- LT_Várzea_Grande___EPE_CN_167284528_138000_CN_32957294_138000/RConn1
  LT_Várzea_Grande___Cristo_Rei_CN_176682224_138000_CN_32957294_138000/RConn2 -- T_32957294__/LConn2 -- LT_Nobres___Várzea_Grande_CN_32957294_138000_CN_169406381_138000/LConn2 -- LT_Várzea_Grande___EPE_CN_167284528_138000_CN_32957294_138000/RConn2
  LT_Várzea_Grande___Cristo_Rei_CN_176682224_138000_CN_32957294_138000/RConn3 -- T_32957294__/LConn3 -- LT_Nobres___Várzea_Grande_CN_32957294_138000_CN_169406381_138000/LConn3 -- bus61/LConn1 -- LT_Várzea_Grande___EPE_CN_167284528_138000_CN_32957294_138000/RConn3
  T_112451827__/LConn1 -- _CN_112451827_138000_CN_111514032_138000/LConn1
  T_112451827__/LConn2 -- _CN_112451827_138000_CN_111514032_138000/LConn2
  _CN_112451827_138000_CN_111514032_138000/LConn3 -- T_112451827__/LConn3 -- bus62/LConn1
  T_111514032__/LConn1 -- _CN_112451827_138000_CN_111514032_138000/RConn1
  T_111514032__/LConn2 -- _CN_112451827_138000_CN_111514032_138000/RConn2
  _CN_112451827_138000_CN_111514032_138000/RConn3 -- T_111514032__/LConn3 -- bus63/LConn1
  T_430385951__Subestação_Guarapuava/LConn1 -- Linha_SE_Guarapuava_SE_Irati_CN_430385951_138000_CN_430390206_138000/RConn1
  T_430385951__Subestação_Guarapuava/LConn2 -- Linha_SE_Guarapuava_SE_Irati_CN_430385951_138000_CN_430390206_138000/RConn2
  Linha_SE_Guarapuava_SE_Irati_CN_430385951_138000_CN_430390206_138000/RConn3 -- T_430385951__Subestação_Guarapuava/LConn3 -- bus64/LConn1
  T_177544973__Subestação_de_Paranatinga/LConn1 -- LT_Primavera_do_Leste___Paranatinga_CN_177544973_138000_CN_177544975_138000/LConn1
  T_177544973__Subestação_de_Paranatinga/LConn2 -- LT_Primavera_do_Leste___Paranatinga_CN_177544973_138000_CN_177544975_138000/LConn2
  LT_Primavera_do_Leste___Paranatinga_CN_177544973_138000_CN_177544975_138000/LConn3 -- T_177544973__Subestação_de_Paranatinga/LConn3 -- bus65/LConn1
  T_177544975__Subestação_Primavera_do_Leste/LConn1 -- LT_Primavera_do_Leste___Paranatinga_CN_177544973_138000_CN_177544975_138000/RConn1
  T_177544975__Subestação_Primavera_do_Leste/LConn2 -- LT_Primavera_do_Leste___Paranatinga_CN_177544973_138000_CN_177544975_138000/RConn2
  LT_Primavera_do_Leste___Paranatinga_CN_177544973_138000_CN_177544975_138000/RConn3 -- T_177544975__Subestação_Primavera_do_Leste/LConn3 -- bus66/LConn1
  _CN_105353506_138000_CN_206109551_138000/LConn1 -- T_105353506_230000_Subestação_Apucarana/RConn1 -- _CN_105353506_138000_CN_396009895_138000/LConn1 -- _CN_105353506_138000_CN_129482585_138000/LConn1 -- L_105353506/LConn1
  _CN_105353506_138000_CN_206109551_138000/LConn2 -- T_105353506_230000_Subestação_Apucarana/RConn2 -- _CN_105353506_138000_CN_396009895_138000/LConn2 -- _CN_105353506_138000_CN_129482585_138000/LConn2 -- L_105353506/LConn2
  _CN_105353506_138000_CN_206109551_138000/LConn3 -- T_105353506_230000_Subestação_Apucarana/RConn3 -- _CN_105353506_138000_CN_396009895_138000/LConn3 -- _CN_105353506_138000_CN_129482585_138000/LConn3 -- L_105353506/LConn3 -- bus67/LConn1
  _CN_105353506_138000_CN_206109551_138000/RConn1 -- T_206109551_230000_Subestação_Sarandi/RConn1 -- L_206109551/LConn1
  _CN_105353506_138000_CN_206109551_138000/RConn2 -- T_206109551_230000_Subestação_Sarandi/RConn2 -- L_206109551/LConn2
  _CN_105353506_138000_CN_206109551_138000/RConn3 -- T_206109551_230000_Subestação_Sarandi/RConn3 -- L_206109551/LConn3 -- bus68/LConn1
  T_396009895_138000_Subestação_Jardim_Tropical/LConn1 -- _CN_105353506_138000_CN_396009895_138000/RConn1
  T_396009895_138000_Subestação_Jardim_Tropical/LConn2 -- _CN_105353506_138000_CN_396009895_138000/RConn2
  _CN_105353506_138000_CN_396009895_138000/RConn3 -- T_396009895_138000_Subestação_Jardim_Tropical/LConn3 -- bus69/LConn1
  _CN_105353506_138000_CN_129482585_138000/RConn1 -- T_129482585_138000_Subestação_Jardim_Alvorada/LConn1 -- _CN_395793739_138000_CN_129482585_138000/LConn1
  _CN_105353506_138000_CN_129482585_138000/RConn2 -- T_129482585_138000_Subestação_Jardim_Alvorada/LConn2 -- _CN_395793739_138000_CN_129482585_138000/LConn2
  _CN_105353506_138000_CN_129482585_138000/RConn3 -- T_129482585_138000_Subestação_Jardim_Alvorada/LConn3 -- _CN_395793739_138000_CN_129482585_138000/LConn3 -- bus70/LConn1
  T_173329706__/LConn1 -- _CN_173329706_138000_CN_215501231_138000/RConn1
  T_173329706__/LConn2 -- _CN_173329706_138000_CN_215501231_138000/RConn2
  _CN_173329706_138000_CN_215501231_138000/RConn3 -- T_173329706__/LConn3 -- bus71/LConn1
  Linha_SE_Ponta_Grossa_Norte_SE_Sabará_CN_306588466_138000_CN_430403964_138000/RConn1 -- T_430403964__Subestação_Sabará/LConn1 -- Linha_SE_Irati_SE_Sabará_CN_430403964_138000_CN_430390206_138000/RConn1
  Linha_SE_Ponta_Grossa_Norte_SE_Sabará_CN_306588466_138000_CN_430403964_138000/RConn2 -- T_430403964__Subestação_Sabará/LConn2 -- Linha_SE_Irati_SE_Sabará_CN_430403964_138000_CN_430390206_138000/RConn2
  Linha_SE_Ponta_Grossa_Norte_SE_Sabará_CN_306588466_138000_CN_430403964_138000/RConn3 -- T_430403964__Subestação_Sabará/LConn3 -- Linha_SE_Irati_SE_Sabará_CN_430403964_138000_CN_430390206_138000/RConn3 -- bus72/LConn1
  T_395653952__Subestação_Barbosa_Ferraz/LConn1 -- _CN_395653952_138000_CN_394083271_138000/RConn1
  T_395653952__Subestação_Barbosa_Ferraz/LConn2 -- _CN_395653952_138000_CN_394083271_138000/RConn2
  _CN_395653952_138000_CN_394083271_138000/RConn3 -- T_395653952__Subestação_Barbosa_Ferraz/LConn3 -- bus73/LConn1
  T_395653957__Subestação_Mamborê/LConn1 -- _CN_395653957_138000_CN_394083271_138000/RConn1
  T_395653957__Subestação_Mamborê/LConn2 -- _CN_395653957_138000_CN_394083271_138000/RConn2
  _CN_395653957_138000_CN_394083271_138000/RConn3 -- T_395653957__Subestação_Mamborê/LConn3 -- bus74/LConn1
  T_395793739_138000_Subestação_Mandacaru/LConn1 -- _CN_395793739_138000_CN_129482585_138000/RConn1
  T_395793739_138000_Subestação_Mandacaru/LConn2 -- _CN_395793739_138000_CN_129482585_138000/RConn2
  _CN_395793739_138000_CN_129482585_138000/RConn3 -- T_395793739_138000_Subestação_Mandacaru/LConn3 -- bus75/LConn1
  T_405782885__Subestação_de_Pombal/LConn1 -- _CN_405782885_138000_CN_398070144_138000/LConn1
  T_405782885__Subestação_de_Pombal/LConn2 -- _CN_405782885_138000_CN_398070144_138000/LConn2
  _CN_405782885_138000_CN_398070144_138000/LConn3 -- T_405782885__Subestação_de_Pombal/LConn3 -- bus76/LConn1
  T_398070144__Subestação_de_Jericó/LConn1 -- _CN_405782885_138000_CN_398070144_138000/RConn1
  T_398070144__Subestação_de_Jericó/LConn2 -- _CN_405782885_138000_CN_398070144_138000/RConn2
  _CN_405782885_138000_CN_398070144_138000/RConn3 -- T_398070144__Subestação_de_Jericó/LConn3 -- bus77/LConn1
  LT_Nobres___Várzea_Grande_CN_32957294_138000_CN_169406381_138000/RConn1 -- T_169406381__Subestação_Trevo_do_Lagarto/RConn1 -- L_169406381/LConn1
  LT_Nobres___Várzea_Grande_CN_32957294_138000_CN_169406381_138000/RConn2 -- T_169406381__Subestação_Trevo_do_Lagarto/RConn2 -- L_169406381/LConn2
  LT_Nobres___Várzea_Grande_CN_32957294_138000_CN_169406381_138000/RConn3 -- T_169406381__Subestação_Trevo_do_Lagarto/RConn3 -- L_169406381/LConn3 -- bus78/LConn1
  T_280699285__/LConn1 -- _CN_280699285_138000_CN_280699287_138000/LConn1
  T_280699285__/LConn2 -- _CN_280699285_138000_CN_280699287_138000/LConn2
  _CN_280699285_138000_CN_280699287_138000/LConn3 -- T_280699285__/LConn3 -- bus79/LConn1
  T_280699287__/LConn1 -- _CN_280699285_138000_CN_280699287_138000/RConn1
  T_280699287__/LConn2 -- _CN_280699285_138000_CN_280699287_138000/RConn2
  _CN_280699285_138000_CN_280699287_138000/RConn3 -- T_280699287__/LConn3 -- bus80/LConn1
  T_122252210__/LConn1 -- _CN_122252210_138000_CN_108224468_138000/RConn1
  T_122252210__/LConn2 -- _CN_122252210_138000_CN_108224468_138000/RConn2
  _CN_122252210_138000_CN_108224468_138000/RConn3 -- T_122252210__/LConn3 -- bus81/LConn1
  T_122252211__/LConn1 -- _CN_122252211_138000_CN_108224468_138000/RConn1
  T_122252211__/LConn2 -- _CN_122252211_138000_CN_108224468_138000/RConn2
  _CN_122252211_138000_CN_108224468_138000/RConn3 -- T_122252211__/LConn3 -- bus82/LConn1
  T_168692185__/LConn1 -- _CN_168692156_138000_CN_168692185_138000/RConn1
  T_168692185__/LConn2 -- _CN_168692156_138000_CN_168692185_138000/RConn2
  _CN_168692156_138000_CN_168692185_138000/RConn3 -- T_168692185__/LConn3 -- bus83/LConn1
  T_108435903__Substação_Frei_Caneca/LConn1 -- _CN_108435903_138000_CN_108224468_138000/RConn1
  T_108435903__Substação_Frei_Caneca/LConn2 -- _CN_108435903_138000_CN_108224468_138000/RConn2
  _CN_108435903_138000_CN_108224468_138000/RConn3 -- T_108435903__Substação_Frei_Caneca/LConn3 -- bus84/LConn1
  LT_Nova_Mutum___Sorriso_C2_CN_312985603_230000_CN_171732983_230000/LConn1 -- T_312985603__Subestação_Nova_Mutum/LConn1 -- LT_Nova_Mutum___Sorriso_C2_CN_312985603_230000_CN_171732980_230000/LConn1
  LT_Nova_Mutum___Sorriso_C2_CN_312985603_230000_CN_171732983_230000/LConn2 -- T_312985603__Subestação_Nova_Mutum/LConn2 -- LT_Nova_Mutum___Sorriso_C2_CN_312985603_230000_CN_171732980_230000/LConn2
  LT_Nova_Mutum___Sorriso_C2_CN_312985603_230000_CN_171732983_230000/LConn3 -- T_312985603__Subestação_Nova_Mutum/LConn3 -- LT_Nova_Mutum___Sorriso_C2_CN_312985603_230000_CN_171732980_230000/LConn3 -- bus85/LConn1
  LT_Nova_Mutum___Sorriso_C2_CN_312985603_230000_CN_171732983_230000/RConn1 -- T_171732983__Subestação_Sorriso/LConn1 -- LT_Nova_Mutum___Sorriso_C1_CN_171732980_230000_CN_171732983_230000/LConn1 -- LT_Sorriso___Sinop_C1_CN_171732982_230000_CN_171732983_230000/LConn1
  LT_Nova_Mutum___Sorriso_C2_CN_312985603_230000_CN_171732983_230000/RConn2 -- T_171732983__Subestação_Sorriso/LConn2 -- LT_Nova_Mutum___Sorriso_C1_CN_171732980_230000_CN_171732983_230000/LConn2 -- LT_Sorriso___Sinop_C1_CN_171732982_230000_CN_171732983_230000/LConn2
  LT_Nova_Mutum___Sorriso_C2_CN_312985603_230000_CN_171732983_230000/RConn3 -- T_171732983__Subestação_Sorriso/LConn3 -- LT_Nova_Mutum___Sorriso_C1_CN_171732980_230000_CN_171732983_230000/LConn3 -- LT_Sorriso___Sinop_C1_CN_171732982_230000_CN_171732983_230000/LConn3 -- bus86/LConn1
  LT_Nova_Mutum___Sorriso_C2_CN_312985603_230000_CN_171732980_230000/RConn1 -- T_171732980__Subestação_Lucas_do_Rio_Verde/LConn1 -- LT_Nova_Mutum___Sorriso_C1_CN_171732980_230000_CN_171732983_230000/RConn1
  LT_Nova_Mutum___Sorriso_C2_CN_312985603_230000_CN_171732980_230000/RConn2 -- T_171732980__Subestação_Lucas_do_Rio_Verde/LConn2 -- LT_Nova_Mutum___Sorriso_C1_CN_171732980_230000_CN_171732983_230000/RConn2
  LT_Nova_Mutum___Sorriso_C2_CN_312985603_230000_CN_171732980_230000/RConn3 -- T_171732980__Subestação_Lucas_do_Rio_Verde/LConn3 -- LT_Nova_Mutum___Sorriso_C1_CN_171732980_230000_CN_171732983_230000/RConn3 -- bus87/LConn1
  _CN_240522248_230000_CN_262122922_230000/LConn1 -- T_240522248__CHESF/LConn1 -- _CN_240522248_230000_CN_262600085_230000/LConn1 -- _CN_240522248_230000_CN_174572759_230000/LConn1 -- _CN_240522248_230000_CN_261953891_230000/LConn1
  _CN_240522248_230000_CN_262122922_230000/LConn2 -- T_240522248__CHESF/LConn2 -- _CN_240522248_230000_CN_262600085_230000/LConn2 -- _CN_240522248_230000_CN_174572759_230000/LConn2 -- _CN_240522248_230000_CN_261953891_230000/LConn2
  _CN_240522248_230000_CN_262122922_230000/LConn3 -- T_240522248__CHESF/LConn3 -- _CN_240522248_230000_CN_262600085_230000/LConn3 -- _CN_240522248_230000_CN_174572759_230000/LConn3 -- _CN_240522248_230000_CN_261953891_230000/LConn3 -- bus88/LConn1
  _CN_240522248_230000_CN_262122922_230000/RConn1 -- T_262122922__Subestação_de_Russas/LConn1 -- _CN_261953891_230000_CN_262122922_230000/LConn1
  _CN_240522248_230000_CN_262122922_230000/RConn2 -- T_262122922__Subestação_de_Russas/LConn2 -- _CN_261953891_230000_CN_262122922_230000/LConn2
  _CN_240522248_230000_CN_262122922_230000/RConn3 -- T_262122922__Subestação_de_Russas/LConn3 -- _CN_261953891_230000_CN_262122922_230000/LConn3 -- bus89/LConn1
  _CN_240522248_230000_CN_262600085_230000/RConn1 -- T_262600085__/RConn1 -- _CN_262608562_230000_CN_262600085_230000/LConn1 -- L_262600085/LConn1
  _CN_240522248_230000_CN_262600085_230000/RConn2 -- T_262600085__/RConn2 -- _CN_262608562_230000_CN_262600085_230000/LConn2 -- L_262600085/LConn2
  _CN_240522248_230000_CN_262600085_230000/RConn3 -- T_262600085__/RConn3 -- _CN_262608562_230000_CN_262600085_230000/LConn3 -- L_262600085/LConn3 -- bus90/LConn1
  _CN_240522248_230000_CN_174572759_230000/RConn1 -- T_174572759__Subestação_Milagres/RConn1 -- L_174572759/LConn1
  _CN_240522248_230000_CN_174572759_230000/RConn2 -- T_174572759__Subestação_Milagres/RConn2 -- L_174572759/LConn2
  _CN_240522248_230000_CN_174572759_230000/RConn3 -- T_174572759__Subestação_Milagres/RConn3 -- L_174572759/LConn3 -- bus91/LConn1
